simulink model "KUKA_LBR_Simulink_model_flatness_based_control"  (R2017a)
(part 18 of 19)

dblCoriolisCentrifugalFullRow7Col4 = (q14*((sin(q1)*sin(q3)*(cos(q4)*cos(q6) + cos(q5)*sin(q4)*sin(q6)) - cos(q1)*(sin(q2)*(cos(q6)*sin(q4) - cos(q4)*cos(q5)*sin(q6)) + cos(q2)*cos(q3)*(cos(q4)*cos(q6) + cos(q5)*sin(q4)*sin(q6))))*(KUKA_LBR_param_.dblLink7InertXX*(cos(q6)*(sin(q1)*sin(q3)*sin(q4) + cos(q1)*(cos(q4)*sin(q2) - cos(q2)*cos(q3)*sin(q4))) - (cos(q5)*(cos(q4)*sin(q1)*sin(q3) - cos(q1)*(cos(q2)*cos(q3)*cos(q4) + sin(q2)*sin(q4))) + (cos(q3)*sin(q1) + cos(q1)*cos(q2)*sin(q3))*sin(q5))*sin(q6)) + KUKA_LBR_param_.dblLink7InertXY*(cos(q6)*(cos(q4)*sin(q1)*sin(q2) - (cos(q2)*cos(q3)*sin(q1) + cos(q1)*sin(q3))*sin(q4)) + (cos(q5)*sin(q1)*sin(q2)*sin(q4) + cos(q1)*(cos(q4)*cos(q5)*sin(q3) + cos(q3)*sin(q5)) + cos(q2)*sin(q1)*(cos(q3)*cos(q4)*cos(q5) - sin(q3)*sin(q5)))*sin(q6)) + KUKA_LBR_param_.dblLink7InertXZ*(cos(q2)*(cos(q4)*cos(q6) + cos(q5)*sin(q4)*sin(q6)) + sin(q2)*(sin(q3)*sin(q5)*sin(q6) + cos(q3)*(cos(q6)*sin(q4) - cos(q4)*cos(q5)*sin(q6))))) + (-(cos(q6)*(cos(q2)*cos(q3)*cos(q4)*sin(q1) + cos(q1)*cos(q4)*sin(q3) + sin(q1)*sin(q2)*sin(q4))) + cos(q5)*(cos(q4)*sin(q1)*sin(q2) - (cos(q2)*cos(q3)*sin(q1) + cos(q1)*sin(q3))*sin(q4))*sin(q6))*(KUKA_LBR_param_.dblLink7InertXY*(cos(q6)*(sin(q1)*sin(q3)*sin(q4) + cos(q1)*(cos(q4)*sin(q2) - cos(q2)*cos(q3)*sin(q4))) - (cos(q5)*(cos(q4)*sin(q1)*sin(q3) - cos(q1)*(cos(q2)*cos(q3)*cos(q4) + sin(q2)*sin(q4))) + (cos(q3)*sin(q1) + cos(q1)*cos(q2)*sin(q3))*sin(q5))*sin(q6)) + KUKA_LBR_param_.dblLink7InertYY*(cos(q6)*(cos(q4)*sin(q1)*sin(q2) - (cos(q2)*cos(q3)*sin(q1) + cos(q1)*sin(q3))*sin(q4)) + (cos(q5)*sin(q1)*sin(q2)*sin(q4) + cos(q1)*(cos(q4)*cos(q5)*sin(q3) + cos(q3)*sin(q5)) + cos(q2)*sin(q1)*(cos(q3)*cos(q4)*cos(q5) - sin(q3)*sin(q5)))*sin(q6)) + KUKA_LBR_param_.dblLink7InertYZ*(cos(q2)*(cos(q4)*cos(q6) + cos(q5)*sin(q4)*sin(q6)) + sin(q2)*(sin(q3)*sin(q5)*sin(q6) + cos(q3)*(cos(q6)*sin(q4) - cos(q4)*cos(q5)*sin(q6))))) + (cos(q2)*(-(cos(q6)*sin(q4)) + cos(q4)*cos(q5)*sin(q6)) + cos(q3)*sin(q2)*(cos(q4)*cos(q6) + cos(q5)*sin(q4)*sin(q6)))*(KUKA_LBR_param_.dblLink7InertXZ*(cos(q6)*(sin(q1)*sin(q3)*sin(q4) + cos(q1)*(cos(q4)*sin(q2) - cos(q2)*cos(q3)*sin(q4))) - (cos(q5)*(cos(q4)*sin(q1)*sin(q3) - cos(q1)*(cos(q2)*cos(q3)*cos(q4) + sin(q2)*sin(q4))) + (cos(q3)*sin(q1) + cos(q1)*cos(q2)*sin(q3))*sin(q5))*sin(q6)) + KUKA_LBR_param_.dblLink7InertYZ*(cos(q6)*(cos(q4)*sin(q1)*sin(q2) - (cos(q2)*cos(q3)*sin(q1) + cos(q1)*sin(q3))*sin(q4)) + (cos(q5)*sin(q1)*sin(q2)*sin(q4) + cos(q1)*(cos(q4)*cos(q5)*sin(q3) + cos(q3)*sin(q5)) + cos(q2)*sin(q1)*(cos(q3)*cos(q4)*cos(q5) - sin(q3)*sin(q5)))*sin(q6)) + KUKA_LBR_param_.dblLink7InertZZ*(cos(q2)*(cos(q4)*cos(q6) + cos(q5)*sin(q4)*sin(q6)) + sin(q2)*(sin(q3)*sin(q5)*sin(q6) + cos(q3)*(cos(q6)*sin(q4) - cos(q4)*cos(q5)*sin(q6))))) + (cos(q6)*(sin(q1)*sin(q3)*sin(q4) + cos(q1)*(cos(q4)*sin(q2) - cos(q2)*cos(q3)*sin(q4))) - (cos(q5)*(cos(q4)*sin(q1)*sin(q3) - cos(q1)*(cos(q2)*cos(q3)*cos(q4) + sin(q2)*sin(q4))) + (cos(q3)*sin(q1) + cos(q1)*cos(q2)*sin(q3))*sin(q5))*sin(q6))*(KUKA_LBR_param_.dblLink7InertXZ*(cos(q2)*(-(cos(q6)*sin(q4)) + cos(q4)*cos(q5)*sin(q6)) + cos(q3)*sin(q2)*(cos(q4)*cos(q6) + cos(q5)*sin(q4)*sin(q6))) - KUKA_LBR_param_.dblLink7InertXY*(sin(q1)*sin(q2)*(cos(q6)*sin(q4) - cos(q4)*cos(q5)*sin(q6)) + cos(q2)*cos(q3)*sin(q1)*(cos(q4)*cos(q6) + cos(q5)*sin(q4)*sin(q6)) + cos(q1)*sin(q3)*(cos(q4)*cos(q6) + cos(q5)*sin(q4)*sin(q6))) + KUKA_LBR_param_.dblLink7InertXX*(sin(q1)*sin(q3)*(cos(q4)*cos(q6) + cos(q5)*sin(q4)*sin(q6)) - cos(q1)*(sin(q2)*(cos(q6)*sin(q4) - cos(q4)*cos(q5)*sin(q6)) + cos(q2)*cos(q3)*(cos(q4)*cos(q6) + cos(q5)*sin(q4)*sin(q6))))) + (cos(q6)*(cos(q4)*sin(q1)*sin(q2) - (cos(q2)*cos(q3)*sin(q1) + cos(q1)*sin(q3))*sin(q4)) + (cos(q5)*sin(q1)*sin(q2)*sin(q4) + cos(q1)*(cos(q4)*cos(q5)*sin(q3) + cos(q3)*sin(q5)) + cos(q2)*sin(q1)*(cos(q3)*cos(q4)*cos(q5) - sin(q3)*sin(q5)))*sin(q6))*(KUKA_LBR_param_.dblLink7InertYZ*(cos(q2)*(-(cos(q6)*sin(q4)) + cos(q4)*cos(q5)*sin(q6)) + cos(q3)*sin(q2)*(cos(q4)*cos(q6) + cos(q5)*sin(q4)*sin(q6))) - KUKA_LBR_param_.dblLink7InertYY*(sin(q1)*sin(q2)*(cos(q6)*sin(q4) - cos(q4)*cos(q5)*sin(q6)) + cos(q2)*cos(q3)*sin(q1)*(cos(q4)*cos(q6) + cos(q5)*sin(q4)*sin(q6)) + cos(q1)*sin(q3)*(cos(q4)*cos(q6) + cos(q5)*sin(q4)*sin(q6))) + KUKA_LBR_param_.dblLink7InertXY*(sin(q1)*sin(q3)*(cos(q4)*cos(q6) + cos(q5)*sin(q4)*sin(q6)) - cos(q1)*(sin(q2)*(cos(q6)*sin(q4) - cos(q4)*cos(q5)*sin(q6)) + cos(q2)*cos(q3)*(cos(q4)*cos(q6) + cos(q5)*sin(q4)*sin(q6))))) + (cos(q2)*(cos(q4)*cos(q6) + cos(q5)*sin(q4)*sin(q6)) + sin(q2)*(sin(q3)*sin(q5)*sin(q6) + cos(q3)*(cos(q6)*sin(q4) - cos(q4)*cos(q5)*sin(q6))))*(KUKA_LBR_param_.dblLink7InertZZ*(cos(q2)*(-(cos(q6)*sin(q4)) + cos(q4)*cos(q5)*sin(q6)) + cos(q3)*sin(q2)*(cos(q4)*cos(q6) + cos(q5)*sin(q4)*sin(q6))) - KUKA_LBR_param_.dblLink7InertYZ*(sin(q1)*sin(q2)*(cos(q6)*sin(q4) - cos(q4)*cos(q5)*sin(q6)) + cos(q2)*cos(q3)*sin(q1)*(cos(q4)*cos(q6) + cos(q5)*sin(q4)*sin(q6)) + cos(q1)*sin(q3)*(cos(q4)*cos(q6) + cos(q5)*sin(q4)*sin(q6))) + KUKA_LBR_param_.dblLink7InertXZ*(sin(q1)*sin(q3)*(cos(q4)*cos(q6) + cos(q5)*sin(q4)*sin(q6)) - cos(q1)*(sin(q2)*(cos(q6)*sin(q4) - cos(q4)*cos(q5)*sin(q6)) + cos(q2)*cos(q3)*(cos(q4)*cos(q6) + cos(q5)*sin(q4)*sin(q6))))) + 2*KUKA_LBR_param_.dblLink7Mass*(cos(q3)*sin(q2)*(-(KUKA_LBR_param_.dblLink7CogX*cos(q7)*sin(q4)*sin(q5)) + KUKA_LBR_param_.dblLink7CogY*cos(q4)*cos(q7)*sin(q6) + KUKA_LBR_param_.dblLink7CogY*sin(q4)*sin(q5)*sin(q7) + KUKA_LBR_param_.dblLink7CogX*cos(q4)*sin(q6)*sin(q7) - cos(q5)*cos(q6)*sin(q4)*(KUKA_LBR_param_.dblLink7CogY*cos(q7) + KUKA_LBR_param_.dblLink7CogX*sin(q7))) - cos(q2)*(sin(q4)*sin(q6)*(KUKA_LBR_param_.dblLink7CogY*cos(q7) + KUKA_LBR_param_.dblLink7CogX*sin(q7)) + cos(q4)*(cos(q5)*cos(q6)*(KUKA_LBR_param_.dblLink7CogY*cos(q7) + KUKA_LBR_param_.dblLink7CogX*sin(q7)) + sin(q5)*(KUKA_LBR_param_.dblLink7CogX*cos(q7) - KUKA_LBR_param_.dblLink7CogY*sin(q7)))))*(-(KUKA_LBR_param_.dblLink7CogY*cos(q6)*cos(q7)*sin(q2)*sin(q3)*sin(q5)) - KUKA_LBR_param_.dblLink7CogX*cos(q2)*cos(q7)*sin(q4)*sin(q5) + KUKA_LBR_param_.dblLink7CogY*cos(q2)*cos(q4)*cos(q7)*sin(q6) - KUKA_LBR_param_.dblLink7CogX*cos(q6)*sin(q2)*sin(q3)*sin(q5)*sin(q7) + KUKA_LBR_param_.dblLink7CogY*cos(q2)*sin(q4)*sin(q5)*sin(q7) + KUKA_LBR_param_.dblLink7CogX*cos(q2)*cos(q4)*sin(q6)*sin(q7) + cos(q5)*(cos(q7)*(KUKA_LBR_param_.dblLink7CogX*sin(q2)*sin(q3) - KUKA_LBR_param_.dblLink7CogY*cos(q2)*cos(q6)*sin(q4)) - (KUKA_LBR_param_.dblLink7CogY*sin(q2)*sin(q3) + KUKA_LBR_param_.dblLink7CogX*cos(q2)*cos(q6)*sin(q4))*sin(q7)) + cos(q3)*sin(q2)*(sin(q4)*sin(q6)*(KUKA_LBR_param_.dblLink7CogY*cos(q7) + KUKA_LBR_param_.dblLink7CogX*sin(q7)) + cos(q4)*(cos(q5)*cos(q6)*(KUKA_LBR_param_.dblLink7CogY*cos(q7) + KUKA_LBR_param_.dblLink7CogX*sin(q7)) + sin(q5)*(KUKA_LBR_param_.dblLink7CogX*cos(q7) - KUKA_LBR_param_.dblLink7CogY*sin(q7))))) + 2*KUKA_LBR_param_.dblLink7Mass*(-(sin(q1)*sin(q3)*(cos(q4)*sin(q6)*(KUKA_LBR_param_.dblLink7CogY*cos(q7) + KUKA_LBR_param_.dblLink7CogX*sin(q7)) - sin(q4)*(cos(q5)*cos(q6)*(KUKA_LBR_param_.dblLink7CogY*cos(q7) + KUKA_LBR_param_.dblLink7CogX*sin(q7)) + sin(q5)*(KUKA_LBR_param_.dblLink7CogX*cos(q7) - KUKA_LBR_param_.dblLink7CogY*sin(q7))))) + cos(q1)*(sin(q2)*(sin(q4)*sin(q6)*(KUKA_LBR_param_.dblLink7CogY*cos(q7) + KUKA_LBR_param_.dblLink7CogX*sin(q7)) + cos(q4)*(cos(q5)*cos(q6)*(KUKA_LBR_param_.dblLink7CogY*cos(q7) + KUKA_LBR_param_.dblLink7CogX*sin(q7)) + sin(q5)*(KUKA_LBR_param_.dblLink7CogX*cos(q7) - KUKA_LBR_param_.dblLink7CogY*sin(q7)))) + cos(q2)*cos(q3)*(cos(q4)*sin(q6)*(KUKA_LBR_param_.dblLink7CogY*cos(q7) + KUKA_LBR_param_.dblLink7CogX*sin(q7)) - sin(q4)*(cos(q5)*cos(q6)*(KUKA_LBR_param_.dblLink7CogY*cos(q7) + KUKA_LBR_param_.dblLink7CogX*sin(q7)) + sin(q5)*(KUKA_LBR_param_.dblLink7CogX*cos(q7) - KUKA_LBR_param_.dblLink7CogY*sin(q7))))))*(sin(q1)*(cos(q3)*(-(cos(q6)*sin(q5)*(KUKA_LBR_param_.dblLink7CogY*cos(q7) + KUKA_LBR_param_.dblLink7CogX*sin(q7))) + cos(q5)*(KUKA_LBR_param_.dblLink7CogX*cos(q7) - KUKA_LBR_param_.dblLink7CogY*sin(q7))) - sin(q3)*(sin(q4)*sin(q6)*(KUKA_LBR_param_.dblLink7CogY*cos(q7) + KUKA_LBR_param_.dblLink7CogX*sin(q7)) + cos(q4)*(cos(q5)*cos(q6)*(KUKA_LBR_param_.dblLink7CogY*cos(q7) + KUKA_LBR_param_.dblLink7CogX*sin(q7)) + sin(q5)*(KUKA_LBR_param_.dblLink7CogX*cos(q7) - KUKA_LBR_param_.dblLink7CogY*sin(q7))))) + cos(q1)*(sin(q2)*(cos(q7)*(KUKA_LBR_param_.dblLink7CogX*sin(q4)*sin(q5) - KUKA_LBR_param_.dblLink7CogY*cos(q4)*sin(q6)) - (KUKA_LBR_param_.dblLink7CogY*sin(q4)*sin(q5) + KUKA_LBR_param_.dblLink7CogX*cos(q4)*sin(q6))*sin(q7) + cos(q5)*cos(q6)*sin(q4)*(KUKA_LBR_param_.dblLink7CogY*cos(q7) + KUKA_LBR_param_.dblLink7CogX*sin(q7))) + cos(q2)*(sin(q3)*(-(cos(q6)*sin(q5)*(KUKA_LBR_param_.dblLink7CogY*cos(q7) + KUKA_LBR_param_.dblLink7CogX*sin(q7))) + cos(q5)*(KUKA_LBR_param_.dblLink7CogX*cos(q7) - KUKA_LBR_param_.dblLink7CogY*sin(q7))) + cos(q3)*(sin(q4)*sin(q6)*(KUKA_LBR_param_.dblLink7CogY*cos(q7) + KUKA_LBR_param_.dblLink7CogX*sin(q7)) + cos(q4)*(cos(q5)*cos(q6)*(KUKA_LBR_param_.dblLink7CogY*cos(q7) + KUKA_LBR_param_.dblLink7CogX*sin(q7)) + sin(q5)*(KUKA_LBR_param_.dblLink7CogX*cos(q7) - KUKA_LBR_param_.dblLink7CogY*sin(q7))))))) + 2*KUKA_LBR_param_.dblLink7Mass*(cos(q1)*sin(q3)*(cos(q4)*sin(q6)*(KUKA_LBR_param_.dblLink7CogY*cos(q7) + KUKA_LBR_param_.dblLink7CogX*sin(q7)) - sin(q4)*(cos(q5)*cos(q6)*(KUKA_LBR_param_.dblLink7CogY*cos(q7) + KUKA_LBR_param_.dblLink7CogX*sin(q7)) + sin(q5)*(KUKA_LBR_param_.dblLink7CogX*cos(q7) - KUKA_LBR_param_.dblLink7CogY*sin(q7)))) + sin(q1)*(sin(q2)*(sin(q4)*sin(q6)*(KUKA_LBR_param_.dblLink7CogY*cos(q7) + KUKA_LBR_param_.dblLink7CogX*sin(q7)) + cos(q4)*(cos(q5)*cos(q6)*(KUKA_LBR_param_.dblLink7CogY*cos(q7) + KUKA_LBR_param_.dblLink7CogX*sin(q7)) + sin(q5)*(KUKA_LBR_param_.dblLink7CogX*cos(q7) - KUKA_LBR_param_.dblLink7CogY*sin(q7)))) + cos(q2)*cos(q3)*(cos(q4)*sin(q6)*(KUKA_LBR_param_.dblLink7CogY*cos(q7) + KUKA_LBR_param_.dblLink7CogX*sin(q7)) - sin(q4)*(cos(q5)*cos(q6)*(KUKA_LBR_param_.dblLink7CogY*cos(q7) + KUKA_LBR_param_.dblLink7CogX*sin(q7)) + sin(q5)*(KUKA_LBR_param_.dblLink7CogX*cos(q7) - KUKA_LBR_param_.dblLink7CogY*sin(q7))))))*(cos(q1)*(cos(q3)*(cos(q6)*sin(q5)*(KUKA_LBR_param_.dblLink7CogY*cos(q7) + KUKA_LBR_param_.dblLink7CogX*sin(q7)) + cos(q5)*(-(KUKA_LBR_param_.dblLink7CogX*cos(q7)) + KUKA_LBR_param_.dblLink7CogY*sin(q7))) + sin(q3)*(sin(q4)*sin(q6)*(KUKA_LBR_param_.dblLink7CogY*cos(q7) + KUKA_LBR_param_.dblLink7CogX*sin(q7)) + cos(q4)*(cos(q5)*cos(q6)*(KUKA_LBR_param_.dblLink7CogY*cos(q7) + KUKA_LBR_param_.dblLink7CogX*sin(q7)) + sin(q5)*(KUKA_LBR_param_.dblLink7CogX*cos(q7) - KUKA_LBR_param_.dblLink7CogY*sin(q7))))) + sin(q1)*(sin(q2)*(cos(q7)*(KUKA_LBR_param_.dblLink7CogX*sin(q4)*sin(q5) - KUKA_LBR_param_.dblLink7CogY*cos(q4)*sin(q6)) - (KUKA_LBR_param_.dblLink7CogY*sin(q4)*sin(q5) + KUKA_LBR_param_.dblLink7CogX*cos(q4)*sin(q6))*sin(q7) + cos(q5)*cos(q6)*sin(q4)*(KUKA_LBR_param_.dblLink7CogY*cos(q7) + KUKA_LBR_param_.dblLink7CogX*sin(q7))) + cos(q2)*(sin(q3)*(-(cos(q6)*sin(q5)*(KUKA_LBR_param_.dblLink7CogY*cos(q7) + KUKA_LBR_param_.dblLink7CogX*sin(q7))) + cos(q5)*(KUKA_LBR_param_.dblLink7CogX*cos(q7) - KUKA_LBR_param_.dblLink7CogY*sin(q7))) + cos(q3)*(sin(q4)*sin(q6)*(KUKA_LBR_param_.dblLink7CogY*cos(q7) + KUKA_LBR_param_.dblLink7CogX*sin(q7)) + cos(q4)*(cos(q5)*cos(q6)*(KUKA_LBR_param_.dblLink7CogY*cos(q7) + KUKA_LBR_param_.dblLink7CogX*sin(q7)) + sin(q5)*(KUKA_LBR_param_.dblLink7CogX*cos(q7) - KUKA_LBR_param_.dblLink7CogY*sin(q7)))))))))/2.0;
dblCoriolisCentrifugalFullRow7Col5 = (q14*(-((KUKA_LBR_param_.dblLink7InertXY*cos(q2)*cos(q5)*sin(q1)*sin(q3) - KUKA_LBR_param_.dblLink7InertXZ*cos(q5)*sin(q2)*sin(q3) - KUKA_LBR_param_.dblLink7InertXX*cos(q4)*sin(q1)*sin(q3)*sin(q5) + KUKA_LBR_param_.dblLink7InertXZ*cos(q2)*sin(q4)*sin(q5) + KUKA_LBR_param_.dblLink7InertXY*sin(q1)*sin(q2)*sin(q4)*sin(q5) + cos(q3)*(KUKA_LBR_param_.dblLink7InertXX*cos(q5)*sin(q1) + cos(q4)*(KUKA_LBR_param_.dblLink7InertXY*cos(q2)*sin(q1) - KUKA_LBR_param_.dblLink7InertXZ*sin(q2))*sin(q5)) + cos(q1)*(KUKA_LBR_param_.dblLink7InertXX*cos(q2)*cos(q5)*sin(q3) + KUKA_LBR_param_.dblLink7InertXY*cos(q4)*sin(q3)*sin(q5) + KUKA_LBR_param_.dblLink7InertXX*sin(q2)*sin(q4)*sin(q5) + cos(q3)*(-(KUKA_LBR_param_.dblLink7InertXY*cos(q5)) + KUKA_LBR_param_.dblLink7InertXX*cos(q2)*cos(q4)*sin(q5))))*sin(q6)*(cos(q6)*(sin(q1)*sin(q3)*sin(q4) + cos(q1)*(cos(q4)*sin(q2) - cos(q2)*cos(q3)*sin(q4))) - (cos(q5)*(cos(q4)*sin(q1)*sin(q3) - cos(q1)*(cos(q2)*cos(q3)*cos(q4) + sin(q2)*sin(q4))) + (cos(q3)*sin(q1) + cos(q1)*cos(q2)*sin(q3))*sin(q5))*sin(q6))) - (KUKA_LBR_param_.dblLink7InertYY*cos(q2)*cos(q5)*sin(q1)*sin(q3) - KUKA_LBR_param_.dblLink7InertYZ*cos(q5)*sin(q2)*sin(q3) - KUKA_LBR_param_.dblLink7InertXY*cos(q4)*sin(q1)*sin(q3)*sin(q5) + KUKA_LBR_param_.dblLink7InertYZ*cos(q2)*sin(q4)*sin(q5) + KUKA_LBR_param_.dblLink7InertYY*sin(q1)*sin(q2)*sin(q4)*sin(q5) + cos(q3)*(KUKA_LBR_param_.dblLink7InertXY*cos(q5)*sin(q1) + cos(q4)*(KUKA_LBR_param_.dblLink7InertYY*cos(q2)*sin(q1) - KUKA_LBR_param_.dblLink7InertYZ*sin(q2))*sin(q5)) + cos(q1)*(KUKA_LBR_param_.dblLink7InertXY*cos(q2)*cos(q5)*sin(q3) + KUKA_LBR_param_.dblLink7InertYY*cos(q4)*sin(q3)*sin(q5) + KUKA_LBR_param_.dblLink7InertXY*sin(q2)*sin(q4)*sin(q5) + cos(q3)*(-(KUKA_LBR_param_.dblLink7InertYY*cos(q5)) + KUKA_LBR_param_.dblLink7InertXY*cos(q2)*cos(q4)*sin(q5))))*sin(q6)*(cos(q6)*(cos(q4)*sin(q1)*sin(q2) - (cos(q2)*cos(q3)*sin(q1) + cos(q1)*sin(q3))*sin(q4)) + (cos(q5)*sin(q1)*sin(q2)*sin(q4) + cos(q1)*(cos(q4)*cos(q5)*sin(q3) + cos(q3)*sin(q5)) + cos(q2)*sin(q1)*(cos(q3)*cos(q4)*cos(q5) - sin(q3)*sin(q5)))*sin(q6)) - (KUKA_LBR_param_.dblLink7InertYZ*cos(q2)*cos(q5)*sin(q1)*sin(q3) - KUKA_LBR_param_.dblLink7InertZZ*cos(q5)*sin(q2)*sin(q3) - KUKA_LBR_param_.dblLink7InertXZ*cos(q4)*sin(q1)*sin(q3)*sin(q5) + KUKA_LBR_param_.dblLink7InertZZ*cos(q2)*sin(q4)*sin(q5) + KUKA_LBR_param_.dblLink7InertYZ*sin(q1)*sin(q2)*sin(q4)*sin(q5) + cos(q3)*(KUKA_LBR_param_.dblLink7InertXZ*cos(q5)*sin(q1) + cos(q4)*(KUKA_LBR_param_.dblLink7InertYZ*cos(q2)*sin(q1) - KUKA_LBR_param_.dblLink7InertZZ*sin(q2))*sin(q5)) + cos(q1)*(KUKA_LBR_param_.dblLink7InertXZ*cos(q2)*cos(q5)*sin(q3) + KUKA_LBR_param_.dblLink7InertYZ*cos(q4)*sin(q3)*sin(q5) + KUKA_LBR_param_.dblLink7InertXZ*sin(q2)*sin(q4)*sin(q5) + cos(q3)*(-(KUKA_LBR_param_.dblLink7InertYZ*cos(q5)) + KUKA_LBR_param_.dblLink7InertXZ*cos(q2)*cos(q4)*sin(q5))))*sin(q6)*(cos(q2)*(cos(q4)*cos(q6) + cos(q5)*sin(q4)*sin(q6)) + sin(q2)*(sin(q3)*sin(q5)*sin(q6) + cos(q3)*(cos(q6)*sin(q4) - cos(q4)*cos(q5)*sin(q6)))) - (-(cos(q4)*sin(q1)*sin(q3)*sin(q5)) + cos(q3)*(cos(q5)*sin(q1) + cos(q1)*cos(q2)*cos(q4)*sin(q5)) + cos(q1)*(cos(q2)*cos(q5)*sin(q3) + sin(q2)*sin(q4)*sin(q5)))*sin(q6)*(KUKA_LBR_param_.dblLink7InertXX*(cos(q6)*(sin(q1)*sin(q3)*sin(q4) + cos(q1)*(cos(q4)*sin(q2) - cos(q2)*cos(q3)*sin(q4))) - (cos(q5)*(cos(q4)*sin(q1)*sin(q3) - cos(q1)*(cos(q2)*cos(q3)*cos(q4) + sin(q2)*sin(q4))) + (cos(q3)*sin(q1) + cos(q1)*cos(q2)*sin(q3))*sin(q5))*sin(q6)) + KUKA_LBR_param_.dblLink7InertXY*(cos(q6)*(cos(q4)*sin(q1)*sin(q2) - (cos(q2)*cos(q3)*sin(q1) + cos(q1)*sin(q3))*sin(q4)) + (cos(q5)*sin(q1)*sin(q2)*sin(q4) + cos(q1)*(cos(q4)*cos(q5)*sin(q3) + cos(q3)*sin(q5)) + cos(q2)*sin(q1)*(cos(q3)*cos(q4)*cos(q5) - sin(q3)*sin(q5)))*sin(q6)) + KUKA_LBR_param_.dblLink7InertXZ*(cos(q2)*(cos(q4)*cos(q6) + cos(q5)*sin(q4)*sin(q6)) + sin(q2)*(sin(q3)*sin(q5)*sin(q6) + cos(q3)*(cos(q6)*sin(q4) - cos(q4)*cos(q5)*sin(q6))))) + (cos(q1)*(cos(q3)*cos(q5) - cos(q4)*sin(q3)*sin(q5)) - sin(q1)*(sin(q2)*sin(q4)*sin(q5) + cos(q2)*(cos(q5)*sin(q3) + cos(q3)*cos(q4)*sin(q5))))*sin(q6)*(KUKA_LBR_param_.dblLink7InertXY*(cos(q6)*(sin(q1)*sin(q3)*sin(q4) + cos(q1)*(cos(q4)*sin(q2) - cos(q2)*cos(q3)*sin(q4))) - (cos(q5)*(cos(q4)*sin(q1)*sin(q3) - cos(q1)*(cos(q2)*cos(q3)*cos(q4) + sin(q2)*sin(q4))) + (cos(q3)*sin(q1) + cos(q1)*cos(q2)*sin(q3))*sin(q5))*sin(q6)) + KUKA_LBR_param_.dblLink7InertYY*(cos(q6)*(cos(q4)*sin(q1)*sin(q2) - (cos(q2)*cos(q3)*sin(q1) + cos(q1)*sin(q3))*sin(q4)) + (cos(q5)*sin(q1)*sin(q2)*sin(q4) + cos(q1)*(cos(q4)*cos(q5)*sin(q3) + cos(q3)*sin(q5)) + cos(q2)*sin(q1)*(cos(q3)*cos(q4)*cos(q5) - sin(q3)*sin(q5)))*sin(q6)) + KUKA_LBR_param_.dblLink7InertYZ*(cos(q2)*(cos(q4)*cos(q6) + cos(q5)*sin(q4)*sin(q6)) + sin(q2)*(sin(q3)*sin(q5)*sin(q6) + cos(q3)*(cos(q6)*sin(q4) - cos(q4)*cos(q5)*sin(q6))))) + (cos(q5)*sin(q2)*sin(q3) + (cos(q3)*cos(q4)*sin(q2) - cos(q2)*sin(q4))*sin(q5))*sin(q6)*(KUKA_LBR_param_.dblLink7InertXZ*(cos(q6)*(sin(q1)*sin(q3)*sin(q4) + cos(q1)*(cos(q4)*sin(q2) - cos(q2)*cos(q3)*sin(q4))) - (cos(q5)*(cos(q4)*sin(q1)*sin(q3) - cos(q1)*(cos(q2)*cos(q3)*cos(q4) + sin(q2)*sin(q4))) + (cos(q3)*sin(q1) + cos(q1)*cos(q2)*sin(q3))*sin(q5))*sin(q6)) + KUKA_LBR_param_.dblLink7InertYZ*(cos(q6)*(cos(q4)*sin(q1)*sin(q2) - (cos(q2)*cos(q3)*sin(q1) + cos(q1)*sin(q3))*sin(q4)) + (cos(q5)*sin(q1)*sin(q2)*sin(q4) + cos(q1)*(cos(q4)*cos(q5)*sin(q3) + cos(q3)*sin(q5)) + cos(q2)*sin(q1)*(cos(q3)*cos(q4)*cos(q5) - sin(q3)*sin(q5)))*sin(q6)) + KUKA_LBR_param_.dblLink7InertZZ*(cos(q2)*(cos(q4)*cos(q6) + cos(q5)*sin(q4)*sin(q6)) + sin(q2)*(sin(q3)*sin(q5)*sin(q6) + cos(q3)*(cos(q6)*sin(q4) - cos(q4)*cos(q5)*sin(q6))))) + 2*KUKA_LBR_param_.dblLink7Mass*(sin(q5)*(cos(q7)*(-(KUKA_LBR_param_.dblLink7CogX*sin(q2)*sin(q3)) + KUKA_LBR_param_.dblLink7CogY*cos(q2)*cos(q6)*sin(q4)) + (KUKA_LBR_param_.dblLink7CogY*sin(q2)*sin(q3) + KUKA_LBR_param_.dblLink7CogX*cos(q2)*cos(q6)*sin(q4))*sin(q7)) + cos(q3)*cos(q4)*sin(q2)*(-(cos(q6)*sin(q5)*(KUKA_LBR_param_.dblLink7CogY*cos(q7) + KUKA_LBR_param_.dblLink7CogX*sin(q7))) + cos(q5)*(KUKA_LBR_param_.dblLink7CogX*cos(q7) - KUKA_LBR_param_.dblLink7CogY*sin(q7))) - cos(q5)*(cos(q6)*sin(q2)*sin(q3)*(KUKA_LBR_param_.dblLink7CogY*cos(q7) + KUKA_LBR_param_.dblLink7CogX*sin(q7)) + cos(q2)*sin(q4)*(KUKA_LBR_param_.dblLink7CogX*cos(q7) - KUKA_LBR_param_.dblLink7CogY*sin(q7))))*(-(KUKA_LBR_param_.dblLink7CogY*cos(q6)*cos(q7)*sin(q2)*sin(q3)*sin(q5)) - KUKA_LBR_param_.dblLink7CogX*cos(q2)*cos(q7)*sin(q4)*sin(q5) + KUKA_LBR_param_.dblLink7CogY*cos(q2)*cos(q4)*cos(q7)*sin(q6) - KUKA_LBR_param_.dblLink7CogX*cos(q6)*sin(q2)*sin(q3)*sin(q5)*sin(q7) + KUKA_LBR_param_.dblLink7CogY*cos(q2)*sin(q4)*sin(q5)*sin(q7) + KUKA_LBR_param_.dblLink7CogX*cos(q2)*cos(q4)*sin(q6)*sin(q7) + cos(q5)*(cos(q7)*(KUKA_LBR_param_.dblLink7CogX*sin(q2)*sin(q3) - KUKA_LBR_param_.dblLink7CogY*cos(q2)*cos(q6)*sin(q4)) - (KUKA_LBR_param_.dblLink7CogY*sin(q2)*sin(q3) + KUKA_LBR_param_.dblLink7CogX*cos(q2)*cos(q6)*sin(q4))*sin(q7)) + cos(q3)*sin(q2)*(sin(q4)*sin(q6)*(KUKA_LBR_param_.dblLink7CogY*cos(q7) + KUKA_LBR_param_.dblLink7CogX*sin(q7)) + cos(q4)*(cos(q5)*cos(q6)*(KUKA_LBR_param_.dblLink7CogY*cos(q7) + KUKA_LBR_param_.dblLink7CogX*sin(q7)) + sin(q5)*(KUKA_LBR_param_.dblLink7CogX*cos(q7) - KUKA_LBR_param_.dblLink7CogY*sin(q7))))) + 2*KUKA_LBR_param_.dblLink7Mass*(sin(q1)*(-(cos(q3)*(cos(q5)*cos(q6)*(KUKA_LBR_param_.dblLink7CogY*cos(q7) + KUKA_LBR_param_.dblLink7CogX*sin(q7)) + sin(q5)*(KUKA_LBR_param_.dblLink7CogX*cos(q7) - KUKA_LBR_param_.dblLink7CogY*sin(q7)))) + cos(q4)*sin(q3)*(cos(q6)*sin(q5)*(KUKA_LBR_param_.dblLink7CogY*cos(q7) + KUKA_LBR_param_.dblLink7CogX*sin(q7)) + cos(q5)*(-(KUKA_LBR_param_.dblLink7CogX*cos(q7)) + KUKA_LBR_param_.dblLink7CogY*sin(q7)))) + cos(q1)*(sin(q2)*sin(q4)*(-(cos(q6)*sin(q5)*(KUKA_LBR_param_.dblLink7CogY*cos(q7) + KUKA_LBR_param_.dblLink7CogX*sin(q7))) + cos(q5)*(KUKA_LBR_param_.dblLink7CogX*cos(q7) - KUKA_LBR_param_.dblLink7CogY*sin(q7))) + cos(q2)*(cos(q3)*cos(q4)*(-(cos(q6)*sin(q5)*(KUKA_LBR_param_.dblLink7CogY*cos(q7) + KUKA_LBR_param_.dblLink7CogX*sin(q7))) + cos(q5)*(KUKA_LBR_param_.dblLink7CogX*cos(q7) - KUKA_LBR_param_.dblLink7CogY*sin(q7))) - sin(q3)*(cos(q5)*cos(q6)*(KUKA_LBR_param_.dblLink7CogY*cos(q7) + KUKA_LBR_param_.dblLink7CogX*sin(q7)) + sin(q5)*(KUKA_LBR_param_.dblLink7CogX*cos(q7) - KUKA_LBR_param_.dblLink7CogY*sin(q7))))))*(sin(q1)*(cos(q3)*(-(cos(q6)*sin(q5)*(KUKA_LBR_param_.dblLink7CogY*cos(q7) + KUKA_LBR_param_.dblLink7CogX*sin(q7))) + cos(q5)*(KUKA_LBR_param_.dblLink7CogX*cos(q7) - KUKA_LBR_param_.dblLink7CogY*sin(q7))) - sin(q3)*(sin(q4)*sin(q6)*(KUKA_LBR_param_.dblLink7CogY*cos(q7) + KUKA_LBR_param_.dblLink7CogX*sin(q7)) + cos(q4)*(cos(q5)*cos(q6)*(KUKA_LBR_param_.dblLink7CogY*cos(q7) + KUKA_LBR_param_.dblLink7CogX*sin(q7)) + sin(q5)*(KUKA_LBR_param_.dblLink7CogX*cos(q7) - KUKA_LBR_param_.dblLink7CogY*sin(q7))))) + cos(q1)*(sin(q2)*(cos(q7)*(KUKA_LBR_param_.dblLink7CogX*sin(q4)*sin(q5) - KUKA_LBR_param_.dblLink7CogY*cos(q4)*sin(q6)) - (KUKA_LBR_param_.dblLink7CogY*sin(q4)*sin(q5) + KUKA_LBR_param_.dblLink7CogX*cos(q4)*sin(q6))*sin(q7) + cos(q5)*cos(q6)*sin(q4)*(KUKA_LBR_param_.dblLink7CogY*cos(q7) + KUKA_LBR_param_.dblLink7CogX*sin(q7))) + cos(q2)*(sin(q3)*(-(cos(q6)*sin(q5)*(KUKA_LBR_param_.dblLink7CogY*cos(q7) + KUKA_LBR_param_.dblLink7CogX*sin(q7))) + cos(q5)*(KUKA_LBR_param_.dblLink7CogX*cos(q7) - KUKA_LBR_param_.dblLink7CogY*sin(q7))) + cos(q3)*(sin(q4)*sin(q6)*(KUKA_LBR_param_.dblLink7CogY*cos(q7) + KUKA_LBR_param_.dblLink7CogX*sin(q7)) + cos(q4)*(cos(q5)*cos(q6)*(KUKA_LBR_param_.dblLink7CogY*cos(q7) + KUKA_LBR_param_.dblLink7CogX*sin(q7)) + sin(q5)*(KUKA_LBR_param_.dblLink7CogX*cos(q7) - KUKA_LBR_param_.dblLink7CogY*sin(q7))))))) + 2*KUKA_LBR_param_.dblLink7Mass*(cos(q1)*(cos(q4)*sin(q3)*(-(cos(q6)*sin(q5)*(KUKA_LBR_param_.dblLink7CogY*cos(q7) + KUKA_LBR_param_.dblLink7CogX*sin(q7))) + cos(q5)*(KUKA_LBR_param_.dblLink7CogX*cos(q7) - KUKA_LBR_param_.dblLink7CogY*sin(q7))) + cos(q3)*(cos(q5)*cos(q6)*(KUKA_LBR_param_.dblLink7CogY*cos(q7) + KUKA_LBR_param_.dblLink7CogX*sin(q7)) + sin(q5)*(KUKA_LBR_param_.dblLink7CogX*cos(q7) - KUKA_LBR_param_.dblLink7CogY*sin(q7)))) + sin(q1)*(sin(q2)*sin(q4)*(-(cos(q6)*sin(q5)*(KUKA_LBR_param_.dblLink7CogY*cos(q7) + KUKA_LBR_param_.dblLink7CogX*sin(q7))) + cos(q5)*(KUKA_LBR_param_.dblLink7CogX*cos(q7) - KUKA_LBR_param_.dblLink7CogY*sin(q7))) + cos(q2)*(cos(q3)*cos(q4)*(-(cos(q6)*sin(q5)*(KUKA_LBR_param_.dblLink7CogY*cos(q7) + KUKA_LBR_param_.dblLink7CogX*sin(q7))) + cos(q5)*(KUKA_LBR_param_.dblLink7CogX*cos(q7) - KUKA_LBR_param_.dblLink7CogY*sin(q7))) - sin(q3)*(cos(q5)*cos(q6)*(KUKA_LBR_param_.dblLink7CogY*cos(q7) + KUKA_LBR_param_.dblLink7CogX*sin(q7)) + sin(q5)*(KUKA_LBR_param_.dblLink7CogX*cos(q7) - KUKA_LBR_param_.dblLink7CogY*sin(q7))))))*(cos(q1)*(cos(q3)*(cos(q6)*sin(q5)*(KUKA_LBR_param_.dblLink7CogY*cos(q7) + KUKA_LBR_param_.dblLink7CogX*sin(q7)) + cos(q5)*(-(KUKA_LBR_param_.dblLink7CogX*cos(q7)) + KUKA_LBR_param_.dblLink7CogY*sin(q7))) + sin(q3)*(sin(q4)*sin(q6)*(KUKA_LBR_param_.dblLink7CogY*cos(q7) + KUKA_LBR_param_.dblLink7CogX*sin(q7)) + cos(q4)*(cos(q5)*cos(q6)*(KUKA_LBR_param_.dblLink7CogY*cos(q7) + KUKA_LBR_param_.dblLink7CogX*sin(q7)) + sin(q5)*(KUKA_LBR_param_.dblLink7CogX*cos(q7) - KUKA_LBR_param_.dblLink7CogY*sin(q7))))) + sin(q1)*(sin(q2)*(cos(q7)*(KUKA_LBR_param_.dblLink7CogX*sin(q4)*sin(q5) - KUKA_LBR_param_.dblLink7CogY*cos(q4)*sin(q6)) - (KUKA_LBR_param_.dblLink7CogY*sin(q4)*sin(q5) + KUKA_LBR_param_.dblLink7CogX*cos(q4)*sin(q6))*sin(q7) + cos(q5)*cos(q6)*sin(q4)*(KUKA_LBR_param_.dblLink7CogY*cos(q7) + KUKA_LBR_param_.dblLink7CogX*sin(q7))) + cos(q2)*(sin(q3)*(-(cos(q6)*sin(q5)*(KUKA_LBR_param_.dblLink7CogY*cos(q7) + KUKA_LBR_param_.dblLink7CogX*sin(q7))) + cos(q5)*(KUKA_LBR_param_.dblLink7CogX*cos(q7) - KUKA_LBR_param_.dblLink7CogY*sin(q7))) + cos(q3)*(sin(q4)*sin(q6)*(KUKA_LBR_param_.dblLink7CogY*cos(q7) + KUKA_LBR_param_.dblLink7CogX*sin(q7)) + cos(q4)*(cos(q5)*cos(q6)*(KUKA_LBR_param_.dblLink7CogY*cos(q7) + KUKA_LBR_param_.dblLink7CogX*sin(q7)) + sin(q5)*(KUKA_LBR_param_.dblLink7CogX*cos(q7) - KUKA_LBR_param_.dblLink7CogY*sin(q7)))))))))/2.0;
dblCoriolisCentrifugalFullRow7Col6 = (q14*((-(sin(q1)*(cos(q4)*cos(q5)*cos(q6)*sin(q3) + cos(q3)*cos(q6)*sin(q5) + sin(q3)*sin(q4)*sin(q6))) + cos(q1)*(sin(q2)*(cos(q5)*cos(q6)*sin(q4) - cos(q4)*sin(q6)) + cos(q2)*(cos(q3)*cos(q4)*cos(q5)*cos(q6) - cos(q6)*sin(q3)*sin(q5) + cos(q3)*sin(q4)*sin(q6))))*(KUKA_LBR_param_.dblLink7InertXX*(cos(q6)*(sin(q1)*sin(q3)*sin(q4) + cos(q1)*(cos(q4)*sin(q2) - cos(q2)*cos(q3)*sin(q4))) - (cos(q5)*(cos(q4)*sin(q1)*sin(q3) - cos(q1)*(cos(q2)*cos(q3)*cos(q4) + sin(q2)*sin(q4))) + (cos(q3)*sin(q1) + cos(q1)*cos(q2)*sin(q3))*sin(q5))*sin(q6)) + KUKA_LBR_param_.dblLink7InertXY*(cos(q6)*(cos(q4)*sin(q1)*sin(q2) - (cos(q2)*cos(q3)*sin(q1) + cos(q1)*sin(q3))*sin(q4)) + (cos(q5)*sin(q1)*sin(q2)*sin(q4) + cos(q1)*(cos(q4)*cos(q5)*sin(q3) + cos(q3)*sin(q5)) + cos(q2)*sin(q1)*(cos(q3)*cos(q4)*cos(q5) - sin(q3)*sin(q5)))*sin(q6)) + KUKA_LBR_param_.dblLink7InertXZ*(cos(q2)*(cos(q4)*cos(q6) + cos(q5)*sin(q4)*sin(q6)) + sin(q2)*(sin(q3)*sin(q5)*sin(q6) + cos(q3)*(cos(q6)*sin(q4) - cos(q4)*cos(q5)*sin(q6))))) + (sin(q1)*sin(q2)*(cos(q5)*cos(q6)*sin(q4) - cos(q4)*sin(q6)) + cos(q1)*(cos(q4)*cos(q5)*cos(q6)*sin(q3) + cos(q3)*cos(q6)*sin(q5) + sin(q3)*sin(q4)*sin(q6)) + cos(q2)*sin(q1)*(-(cos(q6)*sin(q3)*sin(q5)) + cos(q3)*(cos(q4)*cos(q5)*cos(q6) + sin(q4)*sin(q6))))*(KUKA_LBR_param_.dblLink7InertXY*(cos(q6)*(sin(q1)*sin(q3)*sin(q4) + cos(q1)*(cos(q4)*sin(q2) - cos(q2)*cos(q3)*sin(q4))) - (cos(q5)*(cos(q4)*sin(q1)*sin(q3) - cos(q1)*(cos(q2)*cos(q3)*cos(q4) + sin(q2)*sin(q4))) + (cos(q3)*sin(q1) + cos(q1)*cos(q2)*sin(q3))*sin(q5))*sin(q6)) + KUKA_LBR_param_.dblLink7InertYY*(cos(q6)*(cos(q4)*sin(q1)*sin(q2) - (cos(q2)*cos(q3)*sin(q1) + cos(q1)*sin(q3))*sin(q4)) + (cos(q5)*sin(q1)*sin(q2)*sin(q4) + cos(q1)*(cos(q4)*cos(q5)*sin(q3) + cos(q3)*sin(q5)) + cos(q2)*sin(q1)*(cos(q3)*cos(q4)*cos(q5) - sin(q3)*sin(q5)))*sin(q6)) + KUKA_LBR_param_.dblLink7InertYZ*(cos(q2)*(cos(q4)*cos(q6) + cos(q5)*sin(q4)*sin(q6)) + sin(q2)*(sin(q3)*sin(q5)*sin(q6) + cos(q3)*(cos(q6)*sin(q4) - cos(q4)*cos(q5)*sin(q6))))) + (cos(q6)*sin(q2)*sin(q3)*sin(q5) + cos(q2)*(cos(q5)*cos(q6)*sin(q4) - cos(q4)*sin(q6)) - cos(q3)*sin(q2)*(cos(q4)*cos(q5)*cos(q6) + sin(q4)*sin(q6)))*(KUKA_LBR_param_.dblLink7InertXZ*(cos(q6)*(sin(q1)*sin(q3)*sin(q4) + cos(q1)*(cos(q4)*sin(q2) - cos(q2)*cos(q3)*sin(q4))) - (cos(q5)*(cos(q4)*sin(q1)*sin(q3) - cos(q1)*(cos(q2)*cos(q3)*cos(q4) + sin(q2)*sin(q4))) + (cos(q3)*sin(q1) + cos(q1)*cos(q2)*sin(q3))*sin(q5))*sin(q6)) + KUKA_LBR_param_.dblLink7InertYZ*(cos(q6)*(cos(q4)*sin(q1)*sin(q2) - (cos(q2)*cos(q3)*sin(q1) + cos(q1)*sin(q3))*sin(q4)) + (cos(q5)*sin(q1)*sin(q2)*sin(q4) + cos(q1)*(cos(q4)*cos(q5)*sin(q3) + cos(q3)*sin(q5)) + cos(q2)*sin(q1)*(cos(q3)*cos(q4)*cos(q5) - sin(q3)*sin(q5)))*sin(q6)) + KUKA_LBR_param_.dblLink7InertZZ*(cos(q2)*(cos(q4)*cos(q6) + cos(q5)*sin(q4)*sin(q6)) + sin(q2)*(sin(q3)*sin(q5)*sin(q6) + cos(q3)*(cos(q6)*sin(q4) - cos(q4)*cos(q5)*sin(q6))))) + (cos(q6)*(sin(q1)*sin(q3)*sin(q4) + cos(q1)*(cos(q4)*sin(q2) - cos(q2)*cos(q3)*sin(q4))) - (cos(q5)*(cos(q4)*sin(q1)*sin(q3) - cos(q1)*(cos(q2)*cos(q3)*cos(q4) + sin(q2)*sin(q4))) + (cos(q3)*sin(q1) + cos(q1)*cos(q2)*sin(q3))*sin(q5))*sin(q6))*(KUKA_LBR_param_.dblLink7InertXZ*(cos(q6)*sin(q2)*sin(q3)*sin(q5) + cos(q2)*(cos(q5)*cos(q6)*sin(q4) - cos(q4)*sin(q6)) - cos(q3)*sin(q2)*(cos(q4)*cos(q5)*cos(q6) + sin(q4)*sin(q6))) + KUKA_LBR_param_.dblLink7InertXY*(sin(q1)*sin(q2)*(cos(q5)*cos(q6)*sin(q4) - cos(q4)*sin(q6)) + cos(q1)*(cos(q4)*cos(q5)*cos(q6)*sin(q3) + cos(q3)*cos(q6)*sin(q5) + sin(q3)*sin(q4)*sin(q6)) + cos(q2)*sin(q1)*(-(cos(q6)*sin(q3)*sin(q5)) + cos(q3)*(cos(q4)*cos(q5)*cos(q6) + sin(q4)*sin(q6)))) + KUKA_LBR_param_.dblLink7InertXX*(-(sin(q1)*(cos(q4)*cos(q5)*cos(q6)*sin(q3) + cos(q3)*cos(q6)*sin(q5) + sin(q3)*sin(q4)*sin(q6))) + cos(q1)*(sin(q2)*(cos(q5)*cos(q6)*sin(q4) - cos(q4)*sin(q6)) + cos(q2)*(cos(q3)*cos(q4)*cos(q5)*cos(q6) - cos(q6)*sin(q3)*sin(q5) + cos(q3)*sin(q4)*sin(q6))))) + (cos(q6)*(cos(q4)*sin(q1)*sin(q2) - (cos(q2)*cos(q3)*sin(q1) + cos(q1)*sin(q3))*sin(q4)) + (cos(q5)*sin(q1)*sin(q2)*sin(q4) + cos(q1)*(cos(q4)*cos(q5)*sin(q3) + cos(q3)*sin(q5)) + cos(q2)*sin(q1)*(cos(q3)*cos(q4)*cos(q5) - sin(q3)*sin(q5)))*sin(q6))*(KUKA_LBR_param_.dblLink7InertYZ*(cos(q6)*sin(q2)*sin(q3)*sin(q5) + cos(q2)*(cos(q5)*cos(q6)*sin(q4) - cos(q4)*sin(q6)) - cos(q3)*sin(q2)*(cos(q4)*cos(q5)*cos(q6) + sin(q4)*sin(q6))) + KUKA_LBR_param_.dblLink7InertYY*(sin(q1)*sin(q2)*(cos(q5)*cos(q6)*sin(q4) - cos(q4)*sin(q6)) + cos(q1)*(cos(q4)*cos(q5)*cos(q6)*sin(q3) + cos(q3)*cos(q6)*sin(q5) + sin(q3)*sin(q4)*sin(q6)) + cos(q2)*sin(q1)*(-(cos(q6)*sin(q3)*sin(q5)) + cos(q3)*(cos(q4)*cos(q5)*cos(q6) + sin(q4)*sin(q6)))) + KUKA_LBR_param_.dblLink7InertXY*(-(sin(q1)*(cos(q4)*cos(q5)*cos(q6)*sin(q3) + cos(q3)*cos(q6)*sin(q5) + sin(q3)*sin(q4)*sin(q6))) + cos(q1)*(sin(q2)*(cos(q5)*cos(q6)*sin(q4) - cos(q4)*sin(q6)) + cos(q2)*(cos(q3)*cos(q4)*cos(q5)*cos(q6) - cos(q6)*sin(q3)*sin(q5) + cos(q3)*sin(q4)*sin(q6))))) + (cos(q2)*(cos(q4)*cos(q6) + cos(q5)*sin(q4)*sin(q6)) + sin(q2)*(sin(q3)*sin(q5)*sin(q6) + cos(q3)*(cos(q6)*sin(q4) - cos(q4)*cos(q5)*sin(q6))))*(KUKA_LBR_param_.dblLink7InertZZ*(cos(q6)*sin(q2)*sin(q3)*sin(q5) + cos(q2)*(cos(q5)*cos(q6)*sin(q4) - cos(q4)*sin(q6)) - cos(q3)*sin(q2)*(cos(q4)*cos(q5)*cos(q6) + sin(q4)*sin(q6))) + KUKA_LBR_param_.dblLink7InertYZ*(sin(q1)*sin(q2)*(cos(q5)*cos(q6)*sin(q4) - cos(q4)*sin(q6)) + cos(q1)*(cos(q4)*cos(q5)*cos(q6)*sin(q3) + cos(q3)*cos(q6)*sin(q5) + sin(q3)*sin(q4)*sin(q6)) + cos(q2)*sin(q1)*(-(cos(q6)*sin(q3)*sin(q5)) + cos(q3)*(cos(q4)*cos(q5)*cos(q6) + sin(q4)*sin(q6)))) + KUKA_LBR_param_.dblLink7InertXZ*(-(sin(q1)*(cos(q4)*cos(q5)*cos(q6)*sin(q3) + cos(q3)*cos(q6)*sin(q5) + sin(q3)*sin(q4)*sin(q6))) + cos(q1)*(sin(q2)*(cos(q5)*cos(q6)*sin(q4) - cos(q4)*sin(q6)) + cos(q2)*(cos(q3)*cos(q4)*cos(q5)*cos(q6) - cos(q6)*sin(q3)*sin(q5) + cos(q3)*sin(q4)*sin(q6))))) + 2*KUKA_LBR_param_.dblLink7Mass*(cos(q2)*(cos(q4)*cos(q6) + cos(q5)*sin(q4)*sin(q6)) + sin(q2)*(sin(q3)*sin(q5)*sin(q6) + cos(q3)*(cos(q6)*sin(q4) - cos(q4)*cos(q5)*sin(q6))))*(KUKA_LBR_param_.dblLink7CogY*cos(q7) + KUKA_LBR_param_.dblLink7CogX*sin(q7))*(-(KUKA_LBR_param_.dblLink7CogY*cos(q6)*cos(q7)*sin(q2)*sin(q3)*sin(q5)) - KUKA_LBR_param_.dblLink7CogX*cos(q2)*cos(q7)*sin(q4)*sin(q5) + KUKA_LBR_param_.dblLink7CogY*cos(q2)*cos(q4)*cos(q7)*sin(q6) - KUKA_LBR_param_.dblLink7CogX*cos(q6)*sin(q2)*sin(q3)*sin(q5)*sin(q7) + KUKA_LBR_param_.dblLink7CogY*cos(q2)*sin(q4)*sin(q5)*sin(q7) + KUKA_LBR_param_.dblLink7CogX*cos(q2)*cos(q4)*sin(q6)*sin(q7) + cos(q5)*(cos(q7)*(KUKA_LBR_param_.dblLink7CogX*sin(q2)*sin(q3) - KUKA_LBR_param_.dblLink7CogY*cos(q2)*cos(q6)*sin(q4)) - (KUKA_LBR_param_.dblLink7CogY*sin(q2)*sin(q3) + KUKA_LBR_param_.dblLink7CogX*cos(q2)*cos(q6)*sin(q4))*sin(q7)) + cos(q3)*sin(q2)*(sin(q4)*sin(q6)*(KUKA_LBR_param_.dblLink7CogY*cos(q7) + KUKA_LBR_param_.dblLink7CogX*sin(q7)) + cos(q4)*(cos(q5)*cos(q6)*(KUKA_LBR_param_.dblLink7CogY*cos(q7) + KUKA_LBR_param_.dblLink7CogX*sin(q7)) + sin(q5)*(KUKA_LBR_param_.dblLink7CogX*cos(q7) - KUKA_LBR_param_.dblLink7CogY*sin(q7))))) + 2*KUKA_LBR_param_.dblLink7Mass*(sin(q1)*(-(cos(q6)*sin(q3)*sin(q4)) + (cos(q4)*cos(q5)*sin(q3) + cos(q3)*sin(q5))*sin(q6)) + cos(q1)*(cos(q2)*cos(q3)*cos(q6)*sin(q4) - cos(q5)*sin(q2)*sin(q4)*sin(q6) + cos(q2)*sin(q3)*sin(q5)*sin(q6) - cos(q4)*(cos(q6)*sin(q2) + cos(q2)*cos(q3)*cos(q5)*sin(q6))))*(KUKA_LBR_param_.dblLink7CogY*cos(q7) + KUKA_LBR_param_.dblLink7CogX*sin(q7))*(sin(q1)*(cos(q3)*(-(cos(q6)*sin(q5)*(KUKA_LBR_param_.dblLink7CogY*cos(q7) + KUKA_LBR_param_.dblLink7CogX*sin(q7))) + cos(q5)*(KUKA_LBR_param_.dblLink7CogX*cos(q7) - KUKA_LBR_param_.dblLink7CogY*sin(q7))) - sin(q3)*(sin(q4)*sin(q6)*(KUKA_LBR_param_.dblLink7CogY*cos(q7) + KUKA_LBR_param_.dblLink7CogX*sin(q7)) + cos(q4)*(cos(q5)*cos(q6)*(KUKA_LBR_param_.dblLink7CogY*cos(q7) + KUKA_LBR_param_.dblLink7CogX*sin(q7)) + sin(q5)*(KUKA_LBR_param_.dblLink7CogX*cos(q7) - KUKA_LBR_param_.dblLink7CogY*sin(q7))))) + cos(q1)*(sin(q2)*(cos(q7)*(KUKA_LBR_param_.dblLink7CogX*sin(q4)*sin(q5) - KUKA_LBR_param_.dblLink7CogY*cos(q4)*sin(q6)) - (KUKA_LBR_param_.dblLink7CogY*sin(q4)*sin(q5) + KUKA_LBR_param_.dblLink7CogX*cos(q4)*sin(q6))*sin(q7) + cos(q5)*cos(q6)*sin(q4)*(KUKA_LBR_param_.dblLink7CogY*cos(q7) + KUKA_LBR_param_.dblLink7CogX*sin(q7))) + cos(q2)*(sin(q3)*(-(cos(q6)*sin(q5)*(KUKA_LBR_param_.dblLink7CogY*cos(q7) + KUKA_LBR_param_.dblLink7CogX*sin(q7))) + cos(q5)*(KUKA_LBR_param_.dblLink7CogX*cos(q7) - KUKA_LBR_param_.dblLink7CogY*sin(q7))) + cos(q3)*(sin(q4)*sin(q6)*(KUKA_LBR_param_.dblLink7CogY*cos(q7) + KUKA_LBR_param_.dblLink7CogX*sin(q7)) + cos(q4)*(cos(q5)*cos(q6)*(KUKA_LBR_param_.dblLink7CogY*cos(q7) + KUKA_LBR_param_.dblLink7CogX*sin(q7)) + sin(q5)*(KUKA_LBR_param_.dblLink7CogX*cos(q7) - KUKA_LBR_param_.dblLink7CogY*sin(q7))))))) - 2*KUKA_LBR_param_.dblLink7Mass*(-(cos(q1)*cos(q6)*sin(q3)*sin(q4)) + cos(q5)*sin(q1)*sin(q2)*sin(q4)*sin(q6) + cos(q1)*cos(q3)*sin(q5)*sin(q6) + cos(q4)*(cos(q6)*sin(q1)*sin(q2) + cos(q5)*(cos(q2)*cos(q3)*sin(q1) + cos(q1)*sin(q3))*sin(q6)) - cos(q2)*sin(q1)*(cos(q3)*cos(q6)*sin(q4) + sin(q3)*sin(q5)*sin(q6)))*(KUKA_LBR_param_.dblLink7CogY*cos(q7) + KUKA_LBR_param_.dblLink7CogX*sin(q7))*(cos(q1)*(cos(q3)*(cos(q6)*sin(q5)*(KUKA_LBR_param_.dblLink7CogY*cos(q7) + KUKA_LBR_param_.dblLink7CogX*sin(q7)) + cos(q5)*(-(KUKA_LBR_param_.dblLink7CogX*cos(q7)) + KUKA_LBR_param_.dblLink7CogY*sin(q7))) + sin(q3)*(sin(q4)*sin(q6)*(KUKA_LBR_param_.dblLink7CogY*cos(q7) + KUKA_LBR_param_.dblLink7CogX*sin(q7)) + cos(q4)*(cos(q5)*cos(q6)*(KUKA_LBR_param_.dblLink7CogY*cos(q7) + KUKA_LBR_param_.dblLink7CogX*sin(q7)) + sin(q5)*(KUKA_LBR_param_.dblLink7CogX*cos(q7) - KUKA_LBR_param_.dblLink7CogY*sin(q7))))) + sin(q1)*(sin(q2)*(cos(q7)*(KUKA_LBR_param_.dblLink7CogX*sin(q4)*sin(q5) - KUKA_LBR_param_.dblLink7CogY*cos(q4)*sin(q6)) - (KUKA_LBR_param_.dblLink7CogY*sin(q4)*sin(q5) + KUKA_LBR_param_.dblLink7CogX*cos(q4)*sin(q6))*sin(q7) + cos(q5)*cos(q6)*sin(q4)*(KUKA_LBR_param_.dblLink7CogY*cos(q7) + KUKA_LBR_param_.dblLink7CogX*sin(q7))) + cos(q2)*(sin(q3)*(-(cos(q6)*sin(q5)*(KUKA_LBR_param_.dblLink7CogY*cos(q7) + KUKA_LBR_param_.dblLink7CogX*sin(q7))) + cos(q5)*(KUKA_LBR_param_.dblLink7CogX*cos(q7) - KUKA_LBR_param_.dblLink7CogY*sin(q7))) + cos(q3)*(sin(q4)*sin(q6)*(KUKA_LBR_param_.dblLink7CogY*cos(q7) + KUKA_LBR_param_.dblLink7CogX*sin(q7)) + cos(q4)*(cos(q5)*cos(q6)*(KUKA_LBR_param_.dblLink7CogY*cos(q7) + KUKA_LBR_param_.dblLink7CogX*sin(q7)) + sin(q5)*(KUKA_LBR_param_.dblLink7CogX*cos(q7) - KUKA_LBR_param_.dblLink7CogY*sin(q7)))))))))/2.0;
dblCoriolisCentrifugalFullRow7Col7 = KUKA_LBR_param_.dblLink7Mass*q14*((-(KUKA_LBR_param_.dblLink7CogX*cos(q6)*cos(q7)*sin(q2)*sin(q3)*sin(q5)) + KUKA_LBR_param_.dblLink7CogY*cos(q2)*cos(q7)*sin(q4)*sin(q5) + KUKA_LBR_param_.dblLink7CogX*cos(q2)*cos(q4)*cos(q7)*sin(q6) + KUKA_LBR_param_.dblLink7CogY*cos(q6)*sin(q2)*sin(q3)*sin(q5)*sin(q7) + KUKA_LBR_param_.dblLink7CogX*cos(q2)*sin(q4)*sin(q5)*sin(q7) - KUKA_LBR_param_.dblLink7CogY*cos(q2)*cos(q4)*sin(q6)*sin(q7) - cos(q5)*(KUKA_LBR_param_.dblLink7CogY*cos(q7)*sin(q2)*sin(q3) + KUKA_LBR_param_.dblLink7CogX*cos(q2)*cos(q6)*cos(q7)*sin(q4) + KUKA_LBR_param_.dblLink7CogX*sin(q2)*sin(q3)*sin(q7) - KUKA_LBR_param_.dblLink7CogY*cos(q2)*cos(q6)*sin(q4)*sin(q7)) + cos(q3)*sin(q2)*(sin(q4)*sin(q6)*(KUKA_LBR_param_.dblLink7CogX*cos(q7) - KUKA_LBR_param_.dblLink7CogY*sin(q7)) + cos(q4)*(-(sin(q5)*(KUKA_LBR_param_.dblLink7CogY*cos(q7) + KUKA_LBR_param_.dblLink7CogX*sin(q7))) + cos(q5)*cos(q6)*(KUKA_LBR_param_.dblLink7CogX*cos(q7) - KUKA_LBR_param_.dblLink7CogY*sin(q7)))))*(-(KUKA_LBR_param_.dblLink7CogY*cos(q6)*cos(q7)*sin(q2)*sin(q3)*sin(q5)) - KUKA_LBR_param_.dblLink7CogX*cos(q2)*cos(q7)*sin(q4)*sin(q5) + KUKA_LBR_param_.dblLink7CogY*cos(q2)*cos(q4)*cos(q7)*sin(q6) - KUKA_LBR_param_.dblLink7CogX*cos(q6)*sin(q2)*sin(q3)*sin(q5)*sin(q7) + KUKA_LBR_param_.dblLink7CogY*cos(q2)*sin(q4)*sin(q5)*sin(q7) + KUKA_LBR_param_.dblLink7CogX*cos(q2)*cos(q4)*sin(q6)*sin(q7) + cos(q5)*(cos(q7)*(KUKA_LBR_param_.dblLink7CogX*sin(q2)*sin(q3) - KUKA_LBR_param_.dblLink7CogY*cos(q2)*cos(q6)*sin(q4)) - (KUKA_LBR_param_.dblLink7CogY*sin(q2)*sin(q3) + KUKA_LBR_param_.dblLink7CogX*cos(q2)*cos(q6)*sin(q4))*sin(q7)) + cos(q3)*sin(q2)*(sin(q4)*sin(q6)*(KUKA_LBR_param_.dblLink7CogY*cos(q7) + KUKA_LBR_param_.dblLink7CogX*sin(q7)) + cos(q4)*(cos(q5)*cos(q6)*(KUKA_LBR_param_.dblLink7CogY*cos(q7) + KUKA_LBR_param_.dblLink7CogX*sin(q7)) + sin(q5)*(KUKA_LBR_param_.dblLink7CogX*cos(q7) - KUKA_LBR_param_.dblLink7CogY*sin(q7))))) + (sin(q1)*(-(cos(q3)*(cos(q5)*(KUKA_LBR_param_.dblLink7CogY*cos(q7) + KUKA_LBR_param_.dblLink7CogX*sin(q7)) + cos(q6)*sin(q5)*(KUKA_LBR_param_.dblLink7CogX*cos(q7) - KUKA_LBR_param_.dblLink7CogY*sin(q7)))) + sin(q3)*(sin(q4)*sin(q6)*(-(KUKA_LBR_param_.dblLink7CogX*cos(q7)) + KUKA_LBR_param_.dblLink7CogY*sin(q7)) + cos(q4)*(-(KUKA_LBR_param_.dblLink7CogX*cos(q5)*cos(q6)*cos(q7)) + KUKA_LBR_param_.dblLink7CogY*cos(q7)*sin(q5) + KUKA_LBR_param_.dblLink7CogY*cos(q5)*cos(q6)*sin(q7) + KUKA_LBR_param_.dblLink7CogX*sin(q5)*sin(q7)))) + cos(q1)*(sin(q2)*(-(cos(q7)*(KUKA_LBR_param_.dblLink7CogY*sin(q4)*sin(q5) + KUKA_LBR_param_.dblLink7CogX*cos(q4)*sin(q6))) + (-(KUKA_LBR_param_.dblLink7CogX*sin(q4)*sin(q5)) + KUKA_LBR_param_.dblLink7CogY*cos(q4)*sin(q6))*sin(q7) + cos(q5)*cos(q6)*sin(q4)*(KUKA_LBR_param_.dblLink7CogX*cos(q7) - KUKA_LBR_param_.dblLink7CogY*sin(q7))) + cos(q2)*(-(sin(q3)*(cos(q5)*(KUKA_LBR_param_.dblLink7CogY*cos(q7) + KUKA_LBR_param_.dblLink7CogX*sin(q7)) + cos(q6)*sin(q5)*(KUKA_LBR_param_.dblLink7CogX*cos(q7) - KUKA_LBR_param_.dblLink7CogY*sin(q7)))) + cos(q3)*(sin(q4)*sin(q6)*(KUKA_LBR_param_.dblLink7CogX*cos(q7) - KUKA_LBR_param_.dblLink7CogY*sin(q7)) + cos(q4)*(-(sin(q5)*(KUKA_LBR_param_.dblLink7CogY*cos(q7) + KUKA_LBR_param_.dblLink7CogX*sin(q7))) + cos(q5)*cos(q6)*(KUKA_LBR_param_.dblLink7CogX*cos(q7) - KUKA_LBR_param_.dblLink7CogY*sin(q7)))))))*(sin(q1)*(cos(q3)*(-(cos(q6)*sin(q5)*(KUKA_LBR_param_.dblLink7CogY*cos(q7) + KUKA_LBR_param_.dblLink7CogX*sin(q7))) + cos(q5)*(KUKA_LBR_param_.dblLink7CogX*cos(q7) - KUKA_LBR_param_.dblLink7CogY*sin(q7))) - sin(q3)*(sin(q4)*sin(q6)*(KUKA_LBR_param_.dblLink7CogY*cos(q7) + KUKA_LBR_param_.dblLink7CogX*sin(q7)) + cos(q4)*(cos(q5)*cos(q6)*(KUKA_LBR_param_.dblLink7CogY*cos(q7) + KUKA_LBR_param_.dblLink7CogX*sin(q7)) + sin(q5)*(KUKA_LBR_param_.dblLink7CogX*cos(q7) - KUKA_LBR_param_.dblLink7CogY*sin(q7))))) + cos(q1)*(sin(q2)*(cos(q7)*(KUKA_LBR_param_.dblLink7CogX*sin(q4)*sin(q5) - KUKA_LBR_param_.dblLink7CogY*cos(q4)*sin(q6)) - (KUKA_LBR_param_.dblLink7CogY*sin(q4)*sin(q5) + KUKA_LBR_param_.dblLink7CogX*cos(q4)*sin(q6))*sin(q7) + cos(q5)*cos(q6)*sin(q4)*(KUKA_LBR_param_.dblLink7CogY*cos(q7) + KUKA_LBR_param_.dblLink7CogX*sin(q7))) + cos(q2)*(sin(q3)*(-(cos(q6)*sin(q5)*(KUKA_LBR_param_.dblLink7CogY*cos(q7) + KUKA_LBR_param_.dblLink7CogX*sin(q7))) + cos(q5)*(KUKA_LBR_param_.dblLink7CogX*cos(q7) - KUKA_LBR_param_.dblLink7CogY*sin(q7))) + cos(q3)*(sin(q4)*sin(q6)*(KUKA_LBR_param_.dblLink7CogY*cos(q7) + KUKA_LBR_param_.dblLink7CogX*sin(q7)) + cos(q4)*(cos(q5)*cos(q6)*(KUKA_LBR_param_.dblLink7CogY*cos(q7) + KUKA_LBR_param_.dblLink7CogX*sin(q7)) + sin(q5)*(KUKA_LBR_param_.dblLink7CogX*cos(q7) - KUKA_LBR_param_.dblLink7CogY*sin(q7))))))) + (cos(q1)*(cos(q3)*(cos(q5)*(KUKA_LBR_param_.dblLink7CogY*cos(q7) + KUKA_LBR_param_.dblLink7CogX*sin(q7)) + cos(q6)*sin(q5)*(KUKA_LBR_param_.dblLink7CogX*cos(q7) - KUKA_LBR_param_.dblLink7CogY*sin(q7))) + sin(q3)*(sin(q4)*sin(q6)*(KUKA_LBR_param_.dblLink7CogX*cos(q7) - KUKA_LBR_param_.dblLink7CogY*sin(q7)) + cos(q4)*(-(sin(q5)*(KUKA_LBR_param_.dblLink7CogY*cos(q7) + KUKA_LBR_param_.dblLink7CogX*sin(q7))) + cos(q5)*cos(q6)*(KUKA_LBR_param_.dblLink7CogX*cos(q7) - KUKA_LBR_param_.dblLink7CogY*sin(q7))))) + sin(q1)*(sin(q2)*(-(cos(q7)*(KUKA_LBR_param_.dblLink7CogY*sin(q4)*sin(q5) + KUKA_LBR_param_.dblLink7CogX*cos(q4)*sin(q6))) + (-(KUKA_LBR_param_.dblLink7CogX*sin(q4)*sin(q5)) + KUKA_LBR_param_.dblLink7CogY*cos(q4)*sin(q6))*sin(q7) + cos(q5)*cos(q6)*sin(q4)*(KUKA_LBR_param_.dblLink7CogX*cos(q7) - KUKA_LBR_param_.dblLink7CogY*sin(q7))) + cos(q2)*(-(sin(q3)*(cos(q5)*(KUKA_LBR_param_.dblLink7CogY*cos(q7) + KUKA_LBR_param_.dblLink7CogX*sin(q7)) + cos(q6)*sin(q5)*(KUKA_LBR_param_.dblLink7CogX*cos(q7) - KUKA_LBR_param_.dblLink7CogY*sin(q7)))) + cos(q3)*(sin(q4)*sin(q6)*(KUKA_LBR_param_.dblLink7CogX*cos(q7) - KUKA_LBR_param_.dblLink7CogY*sin(q7)) + cos(q4)*(-(sin(q5)*(KUKA_LBR_param_.dblLink7CogY*cos(q7) + KUKA_LBR_param_.dblLink7CogX*sin(q7))) + cos(q5)*cos(q6)*(KUKA_LBR_param_.dblLink7CogX*cos(q7) - KUKA_LBR_param_.dblLink7CogY*sin(q7)))))))*(cos(q1)*(cos(q3)*(cos(q6)*sin(q5)*(KUKA_LBR_param_.dblLink7CogY*cos(q7) + KUKA_LBR_param_.dblLink7CogX*sin(q7)) + cos(q5)*(-(KUKA_LBR_param_.dblLink7CogX*cos(q7)) + KUKA_LBR_param_.dblLink7CogY*sin(q7))) + sin(q3)*(sin(q4)*sin(q6)*(KUKA_LBR_param_.dblLink7CogY*cos(q7) + KUKA_LBR_param_.dblLink7CogX*sin(q7)) + cos(q4)*(cos(q5)*cos(q6)*(KUKA_LBR_param_.dblLink7CogY*cos(q7) + KUKA_LBR_param_.dblLink7CogX*sin(q7)) + sin(q5)*(KUKA_LBR_param_.dblLink7CogX*cos(q7) - KUKA_LBR_param_.dblLink7CogY*sin(q7))))) + sin(q1)*(sin(q2)*(cos(q7)*(KUKA_LBR_param_.dblLink7CogX*sin(q4)*sin(q5) - KUKA_LBR_param_.dblLink7CogY*cos(q4)*sin(q6)) - (KUKA_LBR_param_.dblLink7CogY*sin(q4)*sin(q5) + KUKA_LBR_param_.dblLink7CogX*cos(q4)*sin(q6))*sin(q7) + cos(q5)*cos(q6)*sin(q4)*(KUKA_LBR_param_.dblLink7CogY*cos(q7) + KUKA_LBR_param_.dblLink7CogX*sin(q7))) + cos(q2)*(sin(q3)*(-(cos(q6)*sin(q5)*(KUKA_LBR_param_.dblLink7CogY*cos(q7) + KUKA_LBR_param_.dblLink7CogX*sin(q7))) + cos(q5)*(KUKA_LBR_param_.dblLink7CogX*cos(q7) - KUKA_LBR_param_.dblLink7CogY*sin(q7))) + cos(q3)*(sin(q4)*sin(q6)*(KUKA_LBR_param_.dblLink7CogY*cos(q7) + KUKA_LBR_param_.dblLink7CogX*sin(q7)) + cos(q4)*(cos(q5)*cos(q6)*(KUKA_LBR_param_.dblLink7CogY*cos(q7) + KUKA_LBR_param_.dblLink7CogX*sin(q7)) + sin(q5)*(KUKA_LBR_param_.dblLink7CogX*cos(q7) - KUKA_LBR_param_.dblLink7CogY*sin(q7))))))));

% vecGravityTor %
dblGravityTorRow1Col1 = 0;
dblGravityTorRow2Col1 = KUKA_LBR_param_.dblGravityAcc*(KUKA_LBR_param_.dblLink2Mass*(KUKA_LBR_param_.dblLink2CogX*cos(q2) - KUKA_LBR_param_.dblLink2CogY*sin(q2)) + KUKA_LBR_param_.dblLink3Mass*(-((KUKA_LBR_param_.dblLink23Len + KUKA_LBR_param_.dblLink3CogZ)*sin(q2)) + cos(q2)*(KUKA_LBR_param_.dblLink3CogX*cos(q3) - KUKA_LBR_param_.dblLink3CogY*sin(q3))) - KUKA_LBR_param_.dblLink4Mass*(sin(q2)*(KUKA_LBR_param_.dblLink23Len - KUKA_LBR_param_.dblLink4CogY*cos(q4) - KUKA_LBR_param_.dblLink4CogX*sin(q4)) + cos(q2)*(KUKA_LBR_param_.dblLink4CogZ*sin(q3) + cos(q3)*(-(KUKA_LBR_param_.dblLink4CogX*cos(q4)) + KUKA_LBR_param_.dblLink4CogY*sin(q4)))) - KUKA_LBR_param_.dblLink5Mass*(sin(q2)*(KUKA_LBR_param_.dblLink23Len + (KUKA_LBR_param_.dblLink45Len + KUKA_LBR_param_.dblLink5CogZ)*cos(q4) - KUKA_LBR_param_.dblLink5CogX*cos(q5)*sin(q4) + KUKA_LBR_param_.dblLink5CogY*sin(q4)*sin(q5)) + cos(q2)*(sin(q3)*(KUKA_LBR_param_.dblLink5CogY*cos(q5) + KUKA_LBR_param_.dblLink5CogX*sin(q5)) - cos(q3)*((KUKA_LBR_param_.dblLink45Len + KUKA_LBR_param_.dblLink5CogZ)*sin(q4) + cos(q4)*(KUKA_LBR_param_.dblLink5CogX*cos(q5) - KUKA_LBR_param_.dblLink5CogY*sin(q5))))) + KUKA_LBR_param_.dblLink6Mass*(-(sin(q2)*(KUKA_LBR_param_.dblLink23Len - KUKA_LBR_param_.dblLink6CogX*cos(q5)*cos(q6)*sin(q4) - KUKA_LBR_param_.dblLink6CogZ*sin(q4)*sin(q5) + KUKA_LBR_param_.dblLink6CogY*cos(q5)*sin(q4)*sin(q6) + cos(q4)*(KUKA_LBR_param_.dblLink45Len + KUKA_LBR_param_.dblLink6CogY*cos(q6) + KUKA_LBR_param_.dblLink6CogX*sin(q6)))) + cos(q2)*(sin(q3)*(KUKA_LBR_param_.dblLink6CogZ*cos(q5) + sin(q5)*(-(KUKA_LBR_param_.dblLink6CogX*cos(q6)) + KUKA_LBR_param_.dblLink6CogY*sin(q6))) + cos(q3)*(sin(q4)*(KUKA_LBR_param_.dblLink45Len + KUKA_LBR_param_.dblLink6CogY*cos(q6) + KUKA_LBR_param_.dblLink6CogX*sin(q6)) + cos(q4)*(KUKA_LBR_param_.dblLink6CogX*cos(q5)*cos(q6) + KUKA_LBR_param_.dblLink6CogZ*sin(q5) - KUKA_LBR_param_.dblLink6CogY*cos(q5)*sin(q6))))) + KUKA_LBR_param_.dblLink7Mass*(-(sin(q2)*(KUKA_LBR_param_.dblLink23Len + KUKA_LBR_param_.dblLink7CogY*cos(q7)*sin(q4)*sin(q5) + KUKA_LBR_param_.dblLink7CogX*sin(q4)*sin(q5)*sin(q7) + cos(q5)*sin(q4)*(-(KUKA_LBR_param_.dblLink7CogX*cos(q6)*cos(q7)) + KUKA_LBR_param_.dblLink7CogZ*sin(q6) + KUKA_LBR_param_.dblLink7CogY*cos(q6)*sin(q7)) + cos(q4)*(KUKA_LBR_param_.dblLink45Len + KUKA_LBR_param_.dblLink7CogZ*cos(q6) + KUKA_LBR_param_.dblLink7CogX*cos(q7)*sin(q6) - KUKA_LBR_param_.dblLink7CogY*sin(q6)*sin(q7)))) + cos(q2)*(-(sin(q3)*(cos(q5)*(KUKA_LBR_param_.dblLink7CogY*cos(q7) + KUKA_LBR_param_.dblLink7CogX*sin(q7)) + sin(q5)*(KUKA_LBR_param_.dblLink7CogX*cos(q6)*cos(q7) - KUKA_LBR_param_.dblLink7CogZ*sin(q6) - KUKA_LBR_param_.dblLink7CogY*cos(q6)*sin(q7)))) + cos(q3)*(sin(q4)*(KUKA_LBR_param_.dblLink45Len + KUKA_LBR_param_.dblLink7CogZ*cos(q6) + KUKA_LBR_param_.dblLink7CogX*cos(q7)*sin(q6) - KUKA_LBR_param_.dblLink7CogY*sin(q6)*sin(q7)) - cos(q4)*(sin(q5)*(KUKA_LBR_param_.dblLink7CogY*cos(q7) + KUKA_LBR_param_.dblLink7CogX*sin(q7)) + cos(q5)*(-(KUKA_LBR_param_.dblLink7CogX*cos(q6)*cos(q7)) + KUKA_LBR_param_.dblLink7CogZ*sin(q6) + KUKA_LBR_param_.dblLink7CogY*cos(q6)*sin(q7)))))));
dblGravityTorRow3Col1 = -(KUKA_LBR_param_.dblGravityAcc*sin(q2)*(cos(q3)*(KUKA_LBR_param_.dblLink3CogY*KUKA_LBR_param_.dblLink3Mass + KUKA_LBR_param_.dblLink4CogZ*KUKA_LBR_param_.dblLink4Mass + cos(q5)*(KUKA_LBR_param_.dblLink5CogY*KUKA_LBR_param_.dblLink5Mass - KUKA_LBR_param_.dblLink6CogZ*KUKA_LBR_param_.dblLink6Mass + KUKA_LBR_param_.dblLink7CogY*KUKA_LBR_param_.dblLink7Mass*cos(q7) + KUKA_LBR_param_.dblLink7CogX*KUKA_LBR_param_.dblLink7Mass*sin(q7)) + sin(q5)*(KUKA_LBR_param_.dblLink5CogX*KUKA_LBR_param_.dblLink5Mass - (KUKA_LBR_param_.dblLink6CogY*KUKA_LBR_param_.dblLink6Mass + KUKA_LBR_param_.dblLink7CogZ*KUKA_LBR_param_.dblLink7Mass)*sin(q6) + cos(q6)*(KUKA_LBR_param_.dblLink6CogX*KUKA_LBR_param_.dblLink6Mass + KUKA_LBR_param_.dblLink7CogX*KUKA_LBR_param_.dblLink7Mass*cos(q7) - KUKA_LBR_param_.dblLink7CogY*KUKA_LBR_param_.dblLink7Mass*sin(q7)))) + sin(q3)*(KUKA_LBR_param_.dblLink3CogX*KUKA_LBR_param_.dblLink3Mass + sin(q4)*(-(KUKA_LBR_param_.dblLink4CogY*KUKA_LBR_param_.dblLink4Mass) + KUKA_LBR_param_.dblLink45Len*KUKA_LBR_param_.dblLink5Mass + KUKA_LBR_param_.dblLink5CogZ*KUKA_LBR_param_.dblLink5Mass + KUKA_LBR_param_.dblLink45Len*KUKA_LBR_param_.dblLink6Mass + KUKA_LBR_param_.dblLink45Len*KUKA_LBR_param_.dblLink7Mass + (KUKA_LBR_param_.dblLink6CogY*KUKA_LBR_param_.dblLink6Mass + KUKA_LBR_param_.dblLink7CogZ*KUKA_LBR_param_.dblLink7Mass)*cos(q6) + sin(q6)*(KUKA_LBR_param_.dblLink6CogX*KUKA_LBR_param_.dblLink6Mass + KUKA_LBR_param_.dblLink7CogX*KUKA_LBR_param_.dblLink7Mass*cos(q7) - KUKA_LBR_param_.dblLink7CogY*KUKA_LBR_param_.dblLink7Mass*sin(q7))) + cos(q4)*(KUKA_LBR_param_.dblLink4CogX*KUKA_LBR_param_.dblLink4Mass - sin(q5)*(KUKA_LBR_param_.dblLink5CogY*KUKA_LBR_param_.dblLink5Mass - KUKA_LBR_param_.dblLink6CogZ*KUKA_LBR_param_.dblLink6Mass + KUKA_LBR_param_.dblLink7CogY*KUKA_LBR_param_.dblLink7Mass*cos(q7) + KUKA_LBR_param_.dblLink7CogX*KUKA_LBR_param_.dblLink7Mass*sin(q7)) + cos(q5)*(KUKA_LBR_param_.dblLink5CogX*KUKA_LBR_param_.dblLink5Mass - (KUKA_LBR_param_.dblLink6CogY*KUKA_LBR_param_.dblLink6Mass + KUKA_LBR_param_.dblLink7CogZ*KUKA_LBR_param_.dblLink7Mass)*sin(q6) + cos(q6)*(KUKA_LBR_param_.dblLink6CogX*KUKA_LBR_param_.dblLink6Mass + KUKA_LBR_param_.dblLink7CogX*KUKA_LBR_param_.dblLink7Mass*cos(q7) - KUKA_LBR_param_.dblLink7CogY*KUKA_LBR_param_.dblLink7Mass*sin(q7)))))));
dblGravityTorRow4Col1 = KUKA_LBR_param_.dblGravityAcc*(cos(q3)*sin(q2)*(cos(q4)*(-(KUKA_LBR_param_.dblLink4CogY*KUKA_LBR_param_.dblLink4Mass) + KUKA_LBR_param_.dblLink45Len*KUKA_LBR_param_.dblLink5Mass + KUKA_LBR_param_.dblLink5CogZ*KUKA_LBR_param_.dblLink5Mass + KUKA_LBR_param_.dblLink45Len*KUKA_LBR_param_.dblLink6Mass + KUKA_LBR_param_.dblLink45Len*KUKA_LBR_param_.dblLink7Mass + (KUKA_LBR_param_.dblLink6CogY*KUKA_LBR_param_.dblLink6Mass + KUKA_LBR_param_.dblLink7CogZ*KUKA_LBR_param_.dblLink7Mass)*cos(q6) + sin(q6)*(KUKA_LBR_param_.dblLink6CogX*KUKA_LBR_param_.dblLink6Mass + KUKA_LBR_param_.dblLink7CogX*KUKA_LBR_param_.dblLink7Mass*cos(q7) - KUKA_LBR_param_.dblLink7CogY*KUKA_LBR_param_.dblLink7Mass*sin(q7))) + sin(q4)*(-(KUKA_LBR_param_.dblLink4CogX*KUKA_LBR_param_.dblLink4Mass) + sin(q5)*(KUKA_LBR_param_.dblLink5CogY*KUKA_LBR_param_.dblLink5Mass - KUKA_LBR_param_.dblLink6CogZ*KUKA_LBR_param_.dblLink6Mass + KUKA_LBR_param_.dblLink7CogY*KUKA_LBR_param_.dblLink7Mass*cos(q7) + KUKA_LBR_param_.dblLink7CogX*KUKA_LBR_param_.dblLink7Mass*sin(q7)) + cos(q5)*(-(KUKA_LBR_param_.dblLink5CogX*KUKA_LBR_param_.dblLink5Mass) + KUKA_LBR_param_.dblLink6CogY*KUKA_LBR_param_.dblLink6Mass*sin(q6) + KUKA_LBR_param_.dblLink7CogZ*KUKA_LBR_param_.dblLink7Mass*sin(q6) - cos(q6)*(KUKA_LBR_param_.dblLink6CogX*KUKA_LBR_param_.dblLink6Mass + KUKA_LBR_param_.dblLink7CogX*KUKA_LBR_param_.dblLink7Mass*cos(q7) - KUKA_LBR_param_.dblLink7CogY*KUKA_LBR_param_.dblLink7Mass*sin(q7))))) - cos(q2)*(sin(q4)*(-(KUKA_LBR_param_.dblLink4CogY*KUKA_LBR_param_.dblLink4Mass) + KUKA_LBR_param_.dblLink45Len*KUKA_LBR_param_.dblLink5Mass + KUKA_LBR_param_.dblLink5CogZ*KUKA_LBR_param_.dblLink5Mass + KUKA_LBR_param_.dblLink45Len*KUKA_LBR_param_.dblLink6Mass + KUKA_LBR_param_.dblLink45Len*KUKA_LBR_param_.dblLink7Mass + (KUKA_LBR_param_.dblLink6CogY*KUKA_LBR_param_.dblLink6Mass + KUKA_LBR_param_.dblLink7CogZ*KUKA_LBR_param_.dblLink7Mass)*cos(q6) + sin(q6)*(KUKA_LBR_param_.dblLink6CogX*KUKA_LBR_param_.dblLink6Mass + KUKA_LBR_param_.dblLink7CogX*KUKA_LBR_param_.dblLink7Mass*cos(q7) - KUKA_LBR_param_.dblLink7CogY*KUKA_LBR_param_.dblLink7Mass*sin(q7))) + cos(q4)*(KUKA_LBR_param_.dblLink4CogX*KUKA_LBR_param_.dblLink4Mass - sin(q5)*(KUKA_LBR_param_.dblLink5CogY*KUKA_LBR_param_.dblLink5Mass - KUKA_LBR_param_.dblLink6CogZ*KUKA_LBR_param_.dblLink6Mass + KUKA_LBR_param_.dblLink7CogY*KUKA_LBR_param_.dblLink7Mass*cos(q7) + KUKA_LBR_param_.dblLink7CogX*KUKA_LBR_param_.dblLink7Mass*sin(q7)) + cos(q5)*(KUKA_LBR_param_.dblLink5CogX*KUKA_LBR_param_.dblLink5Mass - (KUKA_LBR_param_.dblLink6CogY*KUKA_LBR_param_.dblLink6Mass + KUKA_LBR_param_.dblLink7CogZ*KUKA_LBR_param_.dblLink7Mass)*sin(q6) + cos(q6)*(KUKA_LBR_param_.dblLink6CogX*KUKA_LBR_param_.dblLink6Mass + KUKA_LBR_param_.dblLink7CogX*KUKA_LBR_param_.dblLink7Mass*cos(q7) - KUKA_LBR_param_.dblLink7CogY*KUKA_LBR_param_.dblLink7Mass*sin(q7))))));
dblGravityTorRow5Col1 = KUKA_LBR_param_.dblGravityAcc*(cos(q5)*(cos(q2)*sin(q4)*(KUKA_LBR_param_.dblLink5CogY*KUKA_LBR_param_.dblLink5Mass - KUKA_LBR_param_.dblLink6CogZ*KUKA_LBR_param_.dblLink6Mass + KUKA_LBR_param_.dblLink7CogY*KUKA_LBR_param_.dblLink7Mass*cos(q7) + KUKA_LBR_param_.dblLink7CogX*KUKA_LBR_param_.dblLink7Mass*sin(q7)) + sin(q2)*sin(q3)*(-(KUKA_LBR_param_.dblLink5CogX*KUKA_LBR_param_.dblLink5Mass) + KUKA_LBR_param_.dblLink6CogY*KUKA_LBR_param_.dblLink6Mass*sin(q6) + KUKA_LBR_param_.dblLink7CogZ*KUKA_LBR_param_.dblLink7Mass*sin(q6) - cos(q6)*(KUKA_LBR_param_.dblLink6CogX*KUKA_LBR_param_.dblLink6Mass + KUKA_LBR_param_.dblLink7CogX*KUKA_LBR_param_.dblLink7Mass*cos(q7) - KUKA_LBR_param_.dblLink7CogY*KUKA_LBR_param_.dblLink7Mass*sin(q7)))) + sin(q5)*(sin(q2)*sin(q3)*(KUKA_LBR_param_.dblLink5CogY*KUKA_LBR_param_.dblLink5Mass - KUKA_LBR_param_.dblLink6CogZ*KUKA_LBR_param_.dblLink6Mass + KUKA_LBR_param_.dblLink7CogY*KUKA_LBR_param_.dblLink7Mass*cos(q7) + KUKA_LBR_param_.dblLink7CogX*KUKA_LBR_param_.dblLink7Mass*sin(q7)) + cos(q2)*sin(q4)*(KUKA_LBR_param_.dblLink5CogX*KUKA_LBR_param_.dblLink5Mass - (KUKA_LBR_param_.dblLink6CogY*KUKA_LBR_param_.dblLink6Mass + KUKA_LBR_param_.dblLink7CogZ*KUKA_LBR_param_.dblLink7Mass)*sin(q6) + cos(q6)*(KUKA_LBR_param_.dblLink6CogX*KUKA_LBR_param_.dblLink6Mass + KUKA_LBR_param_.dblLink7CogX*KUKA_LBR_param_.dblLink7Mass*cos(q7) - KUKA_LBR_param_.dblLink7CogY*KUKA_LBR_param_.dblLink7Mass*sin(q7)))) - cos(q3)*cos(q4)*sin(q2)*(cos(q5)*(KUKA_LBR_param_.dblLink5CogY*KUKA_LBR_param_.dblLink5Mass - KUKA_LBR_param_.dblLink6CogZ*KUKA_LBR_param_.dblLink6Mass + KUKA_LBR_param_.dblLink7CogY*KUKA_LBR_param_.dblLink7Mass*cos(q7) + KUKA_LBR_param_.dblLink7CogX*KUKA_LBR_param_.dblLink7Mass*sin(q7)) + sin(q5)*(KUKA_LBR_param_.dblLink5CogX*KUKA_LBR_param_.dblLink5Mass - (KUKA_LBR_param_.dblLink6CogY*KUKA_LBR_param_.dblLink6Mass + KUKA_LBR_param_.dblLink7CogZ*KUKA_LBR_param_.dblLink7Mass)*sin(q6) + cos(q6)*(KUKA_LBR_param_.dblLink6CogX*KUKA_LBR_param_.dblLink6Mass + KUKA_LBR_param_.dblLink7CogX*KUKA_LBR_param_.dblLink7Mass*cos(q7) - KUKA_LBR_param_.dblLink7CogY*KUKA_LBR_param_.dblLink7Mass*sin(q7)))));
dblGravityTorRow6Col1 = KUKA_LBR_param_.dblGravityAcc*cos(q2)*(cos(q4)*(-((KUKA_LBR_param_.dblLink6CogY*KUKA_LBR_param_.dblLink6Mass + KUKA_LBR_param_.dblLink7CogZ*KUKA_LBR_param_.dblLink7Mass)*sin(q6)) + cos(q6)*(KUKA_LBR_param_.dblLink6CogX*KUKA_LBR_param_.dblLink6Mass + KUKA_LBR_param_.dblLink7CogX*KUKA_LBR_param_.dblLink7Mass*cos(q7) - KUKA_LBR_param_.dblLink7CogY*KUKA_LBR_param_.dblLink7Mass*sin(q7))) + cos(q5)*sin(q4)*((KUKA_LBR_param_.dblLink6CogY*KUKA_LBR_param_.dblLink6Mass + KUKA_LBR_param_.dblLink7CogZ*KUKA_LBR_param_.dblLink7Mass)*cos(q6) + sin(q6)*(KUKA_LBR_param_.dblLink6CogX*KUKA_LBR_param_.dblLink6Mass + KUKA_LBR_param_.dblLink7CogX*KUKA_LBR_param_.dblLink7Mass*cos(q7) - KUKA_LBR_param_.dblLink7CogY*KUKA_LBR_param_.dblLink7Mass*sin(q7)))) - KUKA_LBR_param_.dblGravityAcc*sin(q2)*(-(sin(q3)*sin(q5)*((KUKA_LBR_param_.dblLink6CogY*KUKA_LBR_param_.dblLink6Mass + KUKA_LBR_param_.dblLink7CogZ*KUKA_LBR_param_.dblLink7Mass)*cos(q6) + sin(q6)*(KUKA_LBR_param_.dblLink6CogX*KUKA_LBR_param_.dblLink6Mass + KUKA_LBR_param_.dblLink7CogX*KUKA_LBR_param_.dblLink7Mass*cos(q7) - KUKA_LBR_param_.dblLink7CogY*KUKA_LBR_param_.dblLink7Mass*sin(q7)))) + cos(q3)*(sin(q4)*((KUKA_LBR_param_.dblLink6CogY*KUKA_LBR_param_.dblLink6Mass + KUKA_LBR_param_.dblLink7CogZ*KUKA_LBR_param_.dblLink7Mass)*sin(q6) - cos(q6)*(KUKA_LBR_param_.dblLink6CogX*KUKA_LBR_param_.dblLink6Mass + KUKA_LBR_param_.dblLink7CogX*KUKA_LBR_param_.dblLink7Mass*cos(q7) - KUKA_LBR_param_.dblLink7CogY*KUKA_LBR_param_.dblLink7Mass*sin(q7))) + cos(q4)*cos(q5)*((KUKA_LBR_param_.dblLink6CogY*KUKA_LBR_param_.dblLink6Mass + KUKA_LBR_param_.dblLink7CogZ*KUKA_LBR_param_.dblLink7Mass)*cos(q6) + sin(q6)*(KUKA_LBR_param_.dblLink6CogX*KUKA_LBR_param_.dblLink6Mass + KUKA_LBR_param_.dblLink7CogX*KUKA_LBR_param_.dblLink7Mass*cos(q7) - KUKA_LBR_param_.dblLink7CogY*KUKA_LBR_param_.dblLink7Mass*sin(q7)))));
dblGravityTorRow7Col1 = KUKA_LBR_param_.dblGravityAcc*KUKA_LBR_param_.dblLink7Mass*(KUKA_LBR_param_.dblLink7CogY*cos(q6)*cos(q7)*sin(q2)*sin(q3)*sin(q5) + KUKA_LBR_param_.dblLink7CogX*cos(q2)*cos(q7)*sin(q4)*sin(q5) - KUKA_LBR_param_.dblLink7CogY*cos(q2)*cos(q4)*cos(q7)*sin(q6) + KUKA_LBR_param_.dblLink7CogX*cos(q6)*sin(q2)*sin(q3)*sin(q5)*sin(q7) - KUKA_LBR_param_.dblLink7CogY*cos(q2)*sin(q4)*sin(q5)*sin(q7) - KUKA_LBR_param_.dblLink7CogX*cos(q2)*cos(q4)*sin(q6)*sin(q7) + cos(q5)*(-(KUKA_LBR_param_.dblLink7CogX*cos(q7)*sin(q2)*sin(q3)) + KUKA_LBR_param_.dblLink7CogY*cos(q2)*cos(q6)*cos(q7)*sin(q4) + KUKA_LBR_param_.dblLink7CogY*sin(q2)*sin(q3)*sin(q7) + KUKA_LBR_param_.dblLink7CogX*cos(q2)*cos(q6)*sin(q4)*sin(q7)) - cos(q3)*sin(q2)*(sin(q4)*sin(q6)*(KUKA_LBR_param_.dblLink7CogY*cos(q7) + KUKA_LBR_param_.dblLink7CogX*sin(q7)) + cos(q4)*(cos(q5)*cos(q6)*(KUKA_LBR_param_.dblLink7CogY*cos(q7) + KUKA_LBR_param_.dblLink7CogX*sin(q7)) + sin(q5)*(KUKA_LBR_param_.dblLink7CogX*cos(q7) - KUKA_LBR_param_.dblLink7CogY*sin(q7)))));

dblMassInertFull = [dblMassInertFullRow1Col1 dblMassInertFullRow1Col2 dblMassInertFullRow1Col3 dblMassInertFullRow1Col4 dblMassInertFullRow1Col5 dblMassInertFullRow1Col6 dblMassInertFullRow1Col7; ...
                            dblMassInertFullRow2Col1 dblMassInertFullRow2Col2 dblMassInertFullRow2Col3 dblMassInertFullRow2Col4 dblMassInertFullRow2Col5 dblMassInertFullRow2Col6 dblMassInertFullRow2Col7; ...
                            dblMassInertFullRow3Col1 dblMassInertFullRow3Col2 dblMassInertFullRow3Col3 dblMassInertFullRow3Col4 dblMassInertFullRow3Col5 dblMassInertFullRow3Col6 dblMassInertFullRow3Col7; ...
                            dblMassInertFullRow4Col1 dblMassInertFullRow4Col2 dblMassInertFullRow4Col3 dblMassInertFullRow4Col4 dblMassInertFullRow4Col5 dblMassInertFullRow4Col6 dblMassInertFullRow4Col7; ...
                            dblMassInertFullRow5Col1 dblMassInertFullRow5Col2 dblMassInertFullRow5Col3 dblMassInertFullRow5Col4 dblMassInertFullRow5Col5 dblMassInertFullRow5Col6 dblMassInertFullRow5Col7; ...
                            dblMassInertFullRow6Col1 dblMassInertFullRow6Col2 dblMassInertFullRow6Col3 dblMassInertFullRow6Col4 dblMassInertFullRow6Col5 dblMassInertFullRow6Col6 dblMassInertFullRow6Col7; ...
                            dblMassInertFullRow7Col1 dblMassInertFullRow7Col2 dblMassInertFullRow7Col3 dblMassInertFullRow7Col4 dblMassInertFullRow7Col5 dblMassInertFullRow7Col6 dblMassInertFullRow7Col7];

dblCoriolisCentrifugalFull = [dblCoriolisCentrifugalFullRow1Col1 dblCoriolisCentrifugalFullRow1Col2 dblCoriolisCentrifugalFullRow1Col3 dblCoriolisCentrifugalFullRow1Col4 dblCoriolisCentrifugalFullRow1Col5 dblCoriolisCentrifugalFullRow1Col6 dblCoriolisCentrifugalFullRow1Col7; ...
                            dblCoriolisCentrifugalFullRow2Col1 dblCoriolisCentrifugalFullRow2Col2 dblCoriolisCentrifugalFullRow2Col3 dblCoriolisCentrifugalFullRow2Col4 dblCoriolisCentrifugalFullRow2Col5 dblCoriolisCentrifugalFullRow2Col6 dblCoriolisCentrifugalFullRow2Col7; ...
                            dblCoriolisCentrifugalFullRow3Col1 dblCoriolisCentrifugalFullRow3Col2 dblCoriolisCentrifugalFullRow3Col3 dblCoriolisCentrifugalFullRow3Col4 dblCoriolisCentrifugalFullRow3Col5 dblCoriolisCentrifugalFullRow3Col6 dblCoriolisCentrifugalFullRow3Col7; ...
                            dblCoriolisCentrifugalFullRow4Col1 dblCoriolisCentrifugalFullRow4Col2 dblCoriolisCentrifugalFullRow4Col3 dblCoriolisCentrifugalFullRow4Col4 dblCoriolisCentrifugalFullRow4Col5 dblCoriolisCentrifugalFullRow4Col6 dblCoriolisCentrifugalFullRow4Col7; ...
                            dblCoriolisCentrifugalFullRow5Col1 dblCoriolisCentrifugalFullRow5Col2 dblCoriolisCentrifugalFullRow5Col3 dblCoriolisCentrifugalFullRow5Col4 dblCoriolisCentrifugalFullRow5Col5 dblCoriolisCentrifugalFullRow5Col6 dblCoriolisCentrifugalFullRow5Col7; ...
                            dblCoriolisCentrifugalFullRow6Col1 dblCoriolisCentrifugalFullRow6Col2 dblCoriolisCentrifugalFullRow6Col3 dblCoriolisCentrifugalFullRow6Col4 dblCoriolisCentrifugalFullRow6Col5 dblCoriolisCentrifugalFullRow6Col6 dblCoriolisCentrifugalFullRow6Col7; ...
                            dblCoriolisCentrifugalFullRow7Col1 dblCoriolisCentrifugalFullRow7Col2 dblCoriolisCentrifugalFullRow7Col3 dblCoriolisCentrifugalFullRow7Col4 dblCoriolisCentrifugalFullRow7Col5 dblCoriolisCentrifugalFullRow7Col6 dblCoriolisCentrifugalFullRow7Col7];
  
                        
 dblGravityTor = [dblGravityTorRow1Col1; dblGravityTorRow2Col1; dblGravityTorRow3Col1; dblGravityTorRow4Col1; dblGravityTorRow5Col1; dblGravityTorRow6Col1; dblGravityTorRow7Col1];
 
 


tau = dblMassInertFull * vecJointAcc_ + dblCoriolisCentrifugalFull * vecJointVel_ + dblGravityTor;
